simulink library "outp"  (R2021b)
(part 6 of 11)

      link override Signal_Limit/_minval: Value=KOUTP_ACCLevelMem57_enum_minval
      link override Signal_Override/_ovrdflg: Value=KOUTP_ACCLevelMem57_enum_ovrdflg
      link override Signal_Override/_ovrdval: Value=KOUTP_ACCLevelMem57_enum_ovrdval
  VBCM_APMDoorControlSta_flg_Inproc : FVT_lib/outp/OverrideAndLimit  SystemSampleTime=-1  VariantActivationTime=update diagram  Latency=0  AutoFrameSizeCalculation=off
      link override Signal_Limit/_maxval: Value=KOUTP_APMDoorControlSta_flg_maxval
      link override Signal_Limit/_minval: Value=KOUTP_APMDoorControlSta_flg_minval
      link override Signal_Override/_ovrdflg: Value=KOUTP_APMDoorControlSta_flg_ovrdflg
      link override Signal_Override/_ovrdval: Value=KOUTP_APMDoorControlSta_flg_ovrdval
  VBCM_APSOpenPTG_flg_Inproc : FVT_lib/outp/OverrideAndLimit  SystemSampleTime=-1  VariantActivationTime=update diagram  Latency=0  AutoFrameSizeCalculation=off
      link override Signal_Limit/_maxval: Value=KOUTP_APSOpenPTG_flg_maxval
      link override Signal_Limit/_minval: Value=KOUTP_APSOpenPTG_flg_minval
      link override Signal_Override/_ovrdflg: Value=KOUTP_APSOpenPTG_flg_ovrdflg
      link override Signal_Override/_ovrdval: Value=KOUTP_APSOpenPTG_flg_ovrdval
  VBCM_ATCtrl_enum_Inproc : FVT_lib/outp/OverrideAndLimit  SystemSampleTime=-1  VariantActivationTime=update diagram  Latency=0  AutoFrameSizeCalculation=off
      link override Signal_Limit/_maxval: Value=KOUTP_ATCtrl_enum_maxval
      link override Signal_Limit/_minval: Value=KOUTP_ATCtrl_enum_minval
      link override Signal_Override/_ovrdflg: Value=KOUTP_ATCtrl_enum_ovrdflg
      link override Signal_Override/_ovrdval: Value=KOUTP_ATCtrl_enum_ovrdval
  VBCM_AllDoorSW_flg_Inproc : FVT_lib/outp/OverrideAndLimit  SystemSampleTime=-1  VariantActivationTime=update diagram  Latency=0  AutoFrameSizeCalculation=off
      link override Signal_Limit/_maxval: Value=KOUTP_AllDoorSW_flg_maxval
      link override Signal_Limit/_minval: Value=KOUTP_AllDoorSW_flg_minval
      link override Signal_Override/_ovrdflg: Value=KOUTP_AllDoorSW_flg_ovrdflg
      link override Signal_Override/_ovrdval: Value=KOUTP_AllDoorSW_flg_ovrdval
  VBCM_AmbBrightSta_enum_Inproc : FVT_lib/outp/OverrideAndLimit  SystemSampleTime=-1  VariantActivationTime=update diagram  Latency=0  AutoFrameSizeCalculation=off
      link override Signal_Limit/_maxval: Value=KOUTP_AmbBrightSta_enum_maxval
      link override Signal_Limit/_minval: Value=KOUTP_AmbBrightSta_enum_minval
      link override Signal_Override/_ovrdflg: Value=KOUTP_AmbBrightSta_enum_ovrdflg
      link override Signal_Override/_ovrdval: Value=KOUTP_AmbBrightSta_enum_ovrdval
  VBCM_AmbBrightnessSta1_enum_Inproc : FVT_lib/outp/OverrideAndLimit  SystemSampleTime=-1  VariantActivationTime=update diagram  Latency=0  AutoFrameSizeCalculation=off
      link override Signal_Limit/_maxval: Value=KOUTP_AmbBrightnessSta1_enum_maxval
      link override Signal_Limit/_minval: Value=KOUTP_AmbBrightnessSta1_enum_minval
      link override Signal_Override/_ovrdflg: Value=KOUTP_AmbBrightnessSta1_enum_ovrdflg
      link override Signal_Override/_ovrdval: Value=KOUTP_AmbBrightnessSta1_enum_ovrdval
  VBCM_AmbBrightnessSta2_enum_Inproc : FVT_lib/outp/OverrideAndLimit  SystemSampleTime=-1  VariantActivationTime=update diagram  Latency=0  AutoFrameSizeCalculation=off
      link override Signal_Limit/_maxval: Value=KOUTP_AmbBrightnessSta2_enum_maxval
      link override Signal_Limit/_minval: Value=KOUTP_AmbBrightnessSta2_enum_minval
      link override Signal_Override/_ovrdflg: Value=KOUTP_AmbBrightnessSta2_enum_ovrdflg
      link override Signal_Override/_ovrdval: Value=KOUTP_AmbBrightnessSta2_enum_ovrdval
  VBCM_AmbBrightnessSta3_enum_Inproc : FVT_lib/outp/OverrideAndLimit  SystemSampleTime=-1  VariantActivationTime=update diagram  Latency=0  AutoFrameSizeCalculation=off
      link override Signal_Limit/_maxval: Value=KOUTP_AmbBrightnessSta3_enum_maxval
      link override Signal_Limit/_minval: Value=KOUTP_AmbBrightnessSta3_enum_minval
      link override Signal_Override/_ovrdflg: Value=KOUTP_AmbBrightnessSta3_enum_ovrdflg
      link override Signal_Override/_ovrdval: Value=KOUTP_AmbBrightnessSta3_enum_ovrdval
  VBCM_AmbBrightnessSta4_enum_Inproc : FVT_lib/outp/OverrideAndLimit  SystemSampleTime=-1  VariantActivationTime=update diagram  Latency=0  AutoFrameSizeCalculation=off
      link override Signal_Limit/_maxval: Value=KOUTP_AmbBrightnessSta4_enum_maxval
      link override Signal_Limit/_minval: Value=KOUTP_AmbBrightnessSta4_enum_minval
      link override Signal_Override/_ovrdflg: Value=KOUTP_AmbBrightnessSta4_enum_ovrdflg
      link override Signal_Override/_ovrdval: Value=KOUTP_AmbBrightnessSta4_enum_ovrdval
  VBCM_AmbBrightnessSta5_enum_Inproc : FVT_lib/outp/OverrideAndLimit  SystemSampleTime=-1  VariantActivationTime=update diagram  Latency=0  AutoFrameSizeCalculation=off
      link override Signal_Limit/_maxval: Value=KOUTP_AmbBrightnessSta5_enum_maxval
      link override Signal_Limit/_minval: Value=KOUTP_AmbBrightnessSta5_enum_minval
      link override Signal_Override/_ovrdflg: Value=KOUTP_AmbBrightnessSta5_enum_ovrdflg
      link override Signal_Override/_ovrdval: Value=KOUTP_AmbBrightnessSta5_enum_ovrdval
  VBCM_AmbBrightnessSta7_enum_Inproc : FVT_lib/outp/OverrideAndLimit  SystemSampleTime=-1  VariantActivationTime=update diagram  Latency=0  AutoFrameSizeCalculation=off
      link override Signal_Limit/_maxval: Value=KOUTP_AmbBrightnessSta7_enum_maxval
      link override Signal_Limit/_minval: Value=KOUTP_AmbBrightnessSta7_enum_minval
      link override Signal_Override/_ovrdflg: Value=KOUTP_AmbBrightnessSta7_enum_ovrdflg
      link override Signal_Override/_ovrdval: Value=KOUTP_AmbBrightnessSta7_enum_ovrdval
  VBCM_AmbColorSta1_enum_Inproc : FVT_lib/outp/OverrideAndLimit  SystemSampleTime=-1  VariantActivationTime=update diagram  Latency=0  AutoFrameSizeCalculation=off
      link override Signal_Limit/_maxval: Value=KOUTP_AmbColorSta1_enum_maxval
      link override Signal_Limit/_minval: Value=KOUTP_AmbColorSta1_enum_minval
      link override Signal_Override/_ovrdflg: Value=KOUTP_AmbColorSta1_enum_ovrdflg
      link override Signal_Override/_ovrdval: Value=KOUTP_AmbColorSta1_enum_ovrdval
  VBCM_AmbColorSta2_enum_Inproc : FVT_lib/outp/OverrideAndLimit  SystemSampleTime=-1  VariantActivationTime=update diagram  Latency=0  AutoFrameSizeCalculation=off
      link override Signal_Limit/_maxval: Value=KOUTP_AmbColorSta2_enum_maxval
      link override Signal_Limit/_minval: Value=KOUTP_AmbColorSta2_enum_minval
      link override Signal_Override/_ovrdflg: Value=KOUTP_AmbColorSta2_enum_ovrdflg
      link override Signal_Override/_ovrdval: Value=KOUTP_AmbColorSta2_enum_ovrdval
  VBCM_AmbColorSta3_enum_Inproc : FVT_lib/outp/OverrideAndLimit  SystemSampleTime=-1  VariantActivationTime=update diagram  Latency=0  AutoFrameSizeCalculation=off
      link override Signal_Limit/_maxval: Value=KOUTP_AmbColorSta3_enum_maxval
      link override Signal_Limit/_minval: Value=KOUTP_AmbColorSta3_enum_minval
      link override Signal_Override/_ovrdflg: Value=KOUTP_AmbColorSta3_enum_ovrdflg
      link override Signal_Override/_ovrdval: Value=KOUTP_AmbColorSta3_enum_ovrdval
  VBCM_AmbColorSta4_enum_Inproc : FVT_lib/outp/OverrideAndLimit  SystemSampleTime=-1  VariantActivationTime=update diagram  Latency=0  AutoFrameSizeCalculation=off
      link override Signal_Limit/_maxval: Value=KOUTP_AmbColorSta4_enum_maxval
      link override Signal_Limit/_minval: Value=KOUTP_AmbColorSta4_enum_minval
      link override Signal_Override/_ovrdflg: Value=KOUTP_AmbColorSta4_enum_ovrdflg
      link override Signal_Override/_ovrdval: Value=KOUTP_AmbColorSta4_enum_ovrdval
  VBCM_AmbColorSta5_enum_Inproc : FVT_lib/outp/OverrideAndLimit  SystemSampleTime=-1  VariantActivationTime=update diagram  Latency=0  AutoFrameSizeCalculation=off
      link override Signal_Limit/_maxval: Value=KOUTP_AmbColorSta5_enum_maxval
      link override Signal_Limit/_minval: Value=KOUTP_AmbColorSta5_enum_minval
      link override Signal_Override/_ovrdflg: Value=KOUTP_AmbColorSta5_enum_ovrdflg
      link override Signal_Override/_ovrdval: Value=KOUTP_AmbColorSta5_enum_ovrdval
  VBCM_AmbColorSta7_enum_Inproc : FVT_lib/outp/OverrideAndLimit  SystemSampleTime=-1  VariantActivationTime=update diagram  Latency=0  AutoFrameSizeCalculation=off
      link override Signal_Limit/_maxval: Value=KOUTP_AmbColorSta7_enum_maxval
      link override Signal_Limit/_minval: Value=KOUTP_AmbColorSta7_enum_minval
      link override Signal_Override/_ovrdflg: Value=KOUTP_AmbColorSta7_enum_ovrdflg
      link override Signal_Override/_ovrdval: Value=KOUTP_AmbColorSta7_enum_ovrdval
  VBCM_AmbColorSta_enum_Inproc : FVT_lib/outp/OverrideAndLimit  SystemSampleTime=-1  VariantActivationTime=update diagram  Latency=0  AutoFrameSizeCalculation=off
      link override Signal_Limit/_maxval: Value=KOUTP_AmbColorSta_enum_maxval
      link override Signal_Limit/_minval: Value=KOUTP_AmbColorSta_enum_minval
      link override Signal_Override/_ovrdflg: Value=KOUTP_AmbColorSta_enum_ovrdflg
      link override Signal_Override/_ovrdval: Value=KOUTP_AmbColorSta_enum_ovrdval
  VBCM_AmbDimENFlash_enum_Inproc : FVT_lib/outp/OverrideAndLimit  SystemSampleTime=-1  VariantActivationTime=update diagram  Latency=0  AutoFrameSizeCalculation=off
      link override Signal_Limit/_maxval: Value=KOUTP_AmbDimENFlash_enum_maxval
      link override Signal_Limit/_minval: Value=KOUTP_AmbDimENFlash_enum_minval
      link override Signal_Override/_ovrdflg: Value=KOUTP_AmbDimENFlash_enum_ovrdflg
      link override Signal_Override/_ovrdval: Value=KOUTP_AmbDimENFlash_enum_ovrdval
  VBCM_AmbDimEN_flg_Inproc : FVT_lib/outp/OverrideAndLimit  SystemSampleTime=-1  VariantActivationTime=update diagram  Latency=0  AutoFrameSizeCalculation=off
      link override Signal_Limit/_maxval: Value=KOUTP_AmbDimEN_flg_maxval
      link override Signal_Limit/_minval: Value=KOUTP_AmbDimEN_flg_minval
      link override Signal_Override/_ovrdflg: Value=KOUTP_AmbDimEN_flg_ovrdflg
      link override Signal_Override/_ovrdval: Value=KOUTP_AmbDimEN_flg_ovrdval
  VBCM_AmbFunENFlash_enum_Inproc : FVT_lib/outp/OverrideAndLimit  SystemSampleTime=-1  VariantActivationTime=update diagram  Latency=0  AutoFrameSizeCalculation=off
      link override Signal_Limit/_maxval: Value=KOUTP_AmbFunENFlash_enum_maxval
      link override Signal_Limit/_minval: Value=KOUTP_AmbFunENFlash_enum_minval
      link override Signal_Override/_ovrdflg: Value=KOUTP_AmbFunENFlash_enum_ovrdflg
      link override Signal_Override/_ovrdval: Value=KOUTP_AmbFunENFlash_enum_ovrdval
  VBCM_AmbFunEN_flg_Inproc : FVT_lib/outp/OverrideAndLimit  SystemSampleTime=-1  VariantActivationTime=update diagram  Latency=0  AutoFrameSizeCalculation=off
      link override Signal_Limit/_maxval: Value=KOUTP_AmbFunEN_flg_maxval
      link override Signal_Limit/_minval: Value=KOUTP_AmbFunEN_flg_minval
      link override Signal_Override/_ovrdflg: Value=KOUTP_AmbFunEN_flg_ovrdflg
      link override Signal_Override/_ovrdval: Value=KOUTP_AmbFunEN_flg_ovrdval
  VBCM_AmbLightBreath1_enum_Inproc : FVT_lib/outp/OverrideAndLimit  SystemSampleTime=-1  VariantActivationTime=update diagram  Latency=0  AutoFrameSizeCalculation=off
      link override Signal_Limit/_maxval: Value=KOUTP_AmbLightBreath1_enum_maxval
      link override Signal_Limit/_minval: Value=KOUTP_AmbLightBreath1_enum_minval
      link override Signal_Override/_ovrdflg: Value=KOUTP_AmbLightBreath1_enum_ovrdflg
      link override Signal_Override/_ovrdval: Value=KOUTP_AmbLightBreath1_enum_ovrdval
  VBCM_AmbLightBreath2_enum_Inproc : FVT_lib/outp/OverrideAndLimit  SystemSampleTime=-1  VariantActivationTime=update diagram  Latency=0  AutoFrameSizeCalculation=off
      link override Signal_Limit/_maxval: Value=KOUTP_AmbLightBreath2_enum_maxval
      link override Signal_Limit/_minval: Value=KOUTP_AmbLightBreath2_enum_minval
      link override Signal_Override/_ovrdflg: Value=KOUTP_AmbLightBreath2_enum_ovrdflg
      link override Signal_Override/_ovrdval: Value=KOUTP_AmbLightBreath2_enum_ovrdval
  VBCM_AmbLightBreath3_enum_Inproc : FVT_lib/outp/OverrideAndLimit  SystemSampleTime=-1  VariantActivationTime=update diagram  Latency=0  AutoFrameSizeCalculation=off
      link override Signal_Limit/_maxval: Value=KOUTP_AmbLightBreath3_enum_maxval
      link override Signal_Limit/_minval: Value=KOUTP_AmbLightBreath3_enum_minval
      link override Signal_Override/_ovrdflg: Value=KOUTP_AmbLightBreath3_enum_ovrdflg
      link override Signal_Override/_ovrdval: Value=KOUTP_AmbLightBreath3_enum_ovrdval
  VBCM_AmbLightBreath4_enum_Inproc : FVT_lib/outp/OverrideAndLimit  SystemSampleTime=-1  VariantActivationTime=update diagram  Latency=0  AutoFrameSizeCalculation=off
      link override Signal_Limit/_maxval: Value=KOUTP_AmbLightBreath4_enum_maxval
      link override Signal_Limit/_minval: Value=KOUTP_AmbLightBreath4_enum_minval
      link override Signal_Override/_ovrdflg: Value=KOUTP_AmbLightBreath4_enum_ovrdflg
      link override Signal_Override/_ovrdval: Value=KOUTP_AmbLightBreath4_enum_ovrdval
  VBCM_AmbLightBreath5_enum_Inproc : FVT_lib/outp/OverrideAndLimit  SystemSampleTime=-1  VariantActivationTime=update diagram  Latency=0  AutoFrameSizeCalculation=off
      link override Signal_Limit/_maxval: Value=KOUTP_AmbLightBreath5_enum_maxval
      link override Signal_Limit/_minval: Value=KOUTP_AmbLightBreath5_enum_minval
      link override Signal_Override/_ovrdflg: Value=KOUTP_AmbLightBreath5_enum_ovrdflg
      link override Signal_Override/_ovrdval: Value=KOUTP_AmbLightBreath5_enum_ovrdval
  VBCM_AmbLightBreath6_enum_Inproc : FVT_lib/outp/OverrideAndLimit  SystemSampleTime=-1  VariantActivationTime=update diagram  Latency=0  AutoFrameSizeCalculation=off
      link override Signal_Limit/_maxval: Value=KOUTP_AmbLightBreath6_enum_maxval
      link override Signal_Limit/_minval: Value=KOUTP_AmbLightBreath6_enum_minval
      link override Signal_Override/_ovrdflg: Value=KOUTP_AmbLightBreath6_enum_ovrdflg
      link override Signal_Override/_ovrdval: Value=KOUTP_AmbLightBreath6_enum_ovrdval
  VBCM_AmbLightBrightness1_enum_Inproc : FVT_lib/outp/OverrideAndLimit  SystemSampleTime=-1  VariantActivationTime=update diagram  Latency=0  AutoFrameSizeCalculation=off
      link override Signal_Limit/_maxval: Value=KOUTP_AmbLightBrightness1_enum_maxval
      link override Signal_Limit/_minval: Value=KOUTP_AmbLightBrightness1_enum_minval
      link override Signal_Override/_ovrdflg: Value=KOUTP_AmbLightBrightness1_enum_ovrdflg
      link override Signal_Override/_ovrdval: Value=KOUTP_AmbLightBrightness1_enum_ovrdval
  VBCM_AmbLightBrightness2_enum_Inproc : FVT_lib/outp/OverrideAndLimit  SystemSampleTime=-1  VariantActivationTime=update diagram  Latency=0  AutoFrameSizeCalculation=off
      link override Signal_Limit/_maxval: Value=KOUTP_AmbLightBrightness2_enum_maxval
      link override Signal_Limit/_minval: Value=KOUTP_AmbLightBrightness2_enum_minval
      link override Signal_Override/_ovrdflg: Value=KOUTP_AmbLightBrightness2_enum_ovrdflg
      link override Signal_Override/_ovrdval: Value=KOUTP_AmbLightBrightness2_enum_ovrdval
  VBCM_AmbLightBrightness3_enum_Inproc : FVT_lib/outp/OverrideAndLimit  SystemSampleTime=-1  VariantActivationTime=update diagram  Latency=0  AutoFrameSizeCalculation=off
      link override Signal_Limit/_maxval: Value=KOUTP_AmbLightBrightness3_enum_maxval
      link override Signal_Limit/_minval: Value=KOUTP_AmbLightBrightness3_enum_minval
      link override Signal_Override/_ovrdflg: Value=KOUTP_AmbLightBrightness3_enum_ovrdflg
      link override Signal_Override/_ovrdval: Value=KOUTP_AmbLightBrightness3_enum_ovrdval
  VBCM_AmbLightBrightness4_enum_Inproc : FVT_lib/outp/OverrideAndLimit  SystemSampleTime=-1  VariantActivationTime=update diagram  Latency=0  AutoFrameSizeCalculation=off
      link override Signal_Limit/_maxval: Value=KOUTP_AmbLightBrightness4_enum_maxval
      link override Signal_Limit/_minval: Value=KOUTP_AmbLightBrightness4_enum_minval
      link override Signal_Override/_ovrdflg: Value=KOUTP_AmbLightBrightness4_enum_ovrdflg
      link override Signal_Override/_ovrdval: Value=KOUTP_AmbLightBrightness4_enum_ovrdval
  VBCM_AmbLightBrightness5_enum_Inproc : FVT_lib/outp/OverrideAndLimit  SystemSampleTime=-1  VariantActivationTime=update diagram  Latency=0  AutoFrameSizeCalculation=off
      link override Signal_Limit/_maxval: Value=KOUTP_AmbLightBrightness5_enum_maxval
      link override Signal_Limit/_minval: Value=KOUTP_AmbLightBrightness5_enum_minval
      link override Signal_Override/_ovrdflg: Value=KOUTP_AmbLightBrightness5_enum_ovrdflg
      link override Signal_Override/_ovrdval: Value=KOUTP_AmbLightBrightness5_enum_ovrdval
  VBCM_AmbLightBrightness6_enum_Inproc : FVT_lib/outp/OverrideAndLimit  SystemSampleTime=-1  VariantActivationTime=update diagram  Latency=0  AutoFrameSizeCalculation=off
      link override Signal_Limit/_maxval: Value=KOUTP_AmbLightBrightness6_enum_maxval
      link override Signal_Limit/_minval: Value=KOUTP_AmbLightBrightness6_enum_minval
      link override Signal_Override/_ovrdflg: Value=KOUTP_AmbLightBrightness6_enum_ovrdflg
      link override Signal_Override/_ovrdval: Value=KOUTP_AmbLightBrightness6_enum_ovrdval
  VBCM_AmbLightColor1_enum_Inproc : FVT_lib/outp/OverrideAndLimit  SystemSampleTime=-1  VariantActivationTime=update diagram  Latency=0  AutoFrameSizeCalculation=off
      link override Signal_Limit/_maxval: Value=KOUTP_AmbLightColor1_enum_maxval
      link override Signal_Limit/_minval: Value=KOUTP_AmbLightColor1_enum_minval
      link override Signal_Override/_ovrdflg: Value=KOUTP_AmbLightColor1_enum_ovrdflg
      link override Signal_Override/_ovrdval: Value=KOUTP_AmbLightColor1_enum_ovrdval
  VBCM_AmbLightColor2_enum_Inproc : FVT_lib/outp/OverrideAndLimit  SystemSampleTime=-1  VariantActivationTime=update diagram  Latency=0  AutoFrameSizeCalculation=off
      link override Signal_Limit/_maxval: Value=KOUTP_AmbLightColor2_enum_maxval
      link override Signal_Limit/_minval: Value=KOUTP_AmbLightColor2_enum_minval
      link override Signal_Override/_ovrdflg: Value=KOUTP_AmbLightColor2_enum_ovrdflg
      link override Signal_Override/_ovrdval: Value=KOUTP_AmbLightColor2_enum_ovrdval
  VBCM_AmbLightColor3_enum_Inproc : FVT_lib/outp/OverrideAndLimit  SystemSampleTime=-1  VariantActivationTime=update diagram  Latency=0  AutoFrameSizeCalculation=off
      link override Signal_Limit/_maxval: Value=KOUTP_AmbLightColor3_enum_maxval
      link override Signal_Limit/_minval: Value=KOUTP_AmbLightColor3_enum_minval
      link override Signal_Override/_ovrdflg: Value=KOUTP_AmbLightColor3_enum_ovrdflg
      link override Signal_Override/_ovrdval: Value=KOUTP_AmbLightColor3_enum_ovrdval
  VBCM_AmbLightColor4_enum_Inproc : FVT_lib/outp/OverrideAndLimit  SystemSampleTime=-1  VariantActivationTime=update diagram  Latency=0  AutoFrameSizeCalculation=off
      link override Signal_Limit/_maxval: Value=KOUTP_AmbLightColor4_enum_maxval
      link override Signal_Limit/_minval: Value=KOUTP_AmbLightColor4_enum_minval
      link override Signal_Override/_ovrdflg: Value=KOUTP_AmbLightColor4_enum_ovrdflg
      link override Signal_Override/_ovrdval: Value=KOUTP_AmbLightColor4_enum_ovrdval
  VBCM_AmbLightColor5_enum_Inproc : FVT_lib/outp/OverrideAndLimit  SystemSampleTime=-1  VariantActivationTime=update diagram  Latency=0  AutoFrameSizeCalculation=off
      link override Signal_Limit/_maxval: Value=KOUTP_AmbLightColor5_enum_maxval
      link override Signal_Limit/_minval: Value=KOUTP_AmbLightColor5_enum_minval
      link override Signal_Override/_ovrdflg: Value=KOUTP_AmbLightColor5_enum_ovrdflg
      link override Signal_Override/_ovrdval: Value=KOUTP_AmbLightColor5_enum_ovrdval
  VBCM_AmbLightColor6_enum_Inproc : FVT_lib/outp/OverrideAndLimit  SystemSampleTime=-1  VariantActivationTime=update diagram  Latency=0  AutoFrameSizeCalculation=off
      link override Signal_Limit/_maxval: Value=KOUTP_AmbLightColor6_enum_maxval
      link override Signal_Limit/_minval: Value=KOUTP_AmbLightColor6_enum_minval
      link override Signal_Override/_ovrdflg: Value=KOUTP_AmbLightColor6_enum_ovrdflg
      link override Signal_Override/_ovrdval: Value=KOUTP_AmbLightColor6_enum_ovrdval
  VBCM_AmbLinkDriStaFlash_enum_Inproc : FVT_lib/outp/OverrideAndLimit  SystemSampleTime=-1  VariantActivationTime=update diagram  Latency=0  AutoFrameSizeCalculation=off
      link override Signal_Limit/_maxval: Value=KOUTP_AmbLinkDriStaFlash_enum_maxval
      link override Signal_Limit/_minval: Value=KOUTP_AmbLinkDriStaFlash_enum_minval
      link override Signal_Override/_ovrdflg: Value=KOUTP_AmbLinkDriStaFlash_enum_ovrdflg
      link override Signal_Override/_ovrdval: Value=KOUTP_AmbLinkDriStaFlash_enum_ovrdval
  VBCM_AmbLinkDriSta_flg_Inproc : FVT_lib/outp/OverrideAndLimit  SystemSampleTime=-1  VariantActivationTime=update diagram  Latency=0  AutoFrameSizeCalculation=off
      link override Signal_Limit/_maxval: Value=KOUTP_AmbLinkDriSta_flg_maxval
      link override Signal_Limit/_minval: Value=KOUTP_AmbLinkDriSta_flg_minval
      link override Signal_Override/_ovrdflg: Value=KOUTP_AmbLinkDriSta_flg_ovrdflg
      link override Signal_Override/_ovrdval: Value=KOUTP_AmbLinkDriSta_flg_ovrdval
  VBCM_AmbODAENFlash_enum_Inproc : FVT_lib/outp/OverrideAndLimit  SystemSampleTime=-1  VariantActivationTime=update diagram  Latency=0  AutoFrameSizeCalculation=off
      link override Signal_Limit/_maxval: Value=KOUTP_AmbODAENFlash_enum_maxval
      link override Signal_Limit/_minval: Value=KOUTP_AmbODAENFlash_enum_minval
      link override Signal_Override/_ovrdflg: Value=KOUTP_AmbODAENFlash_enum_ovrdflg
      link override Signal_Override/_ovrdval: Value=KOUTP_AmbODAENFlash_enum_ovrdval
  VBCM_AmbODAEN_flg_Inproc : FVT_lib/outp/OverrideAndLimit  SystemSampleTime=-1  VariantActivationTime=update diagram  Latency=0  AutoFrameSizeCalculation=off
      link override Signal_Limit/_maxval: Value=KOUTP_AmbODAEN_flg_maxval
      link override Signal_Limit/_minval: Value=KOUTP_AmbODAEN_flg_minval
      link override Signal_Override/_ovrdflg: Value=KOUTP_AmbODAEN_flg_ovrdflg
      link override Signal_Override/_ovrdval: Value=KOUTP_AmbODAEN_flg_ovrdval
  VBCM_AmbPwrWarnENFlash_enum_Inproc : FVT_lib/outp/OverrideAndLimit  SystemSampleTime=-1  VariantActivationTime=update diagram  Latency=0  AutoFrameSizeCalculation=off
      link override Signal_Limit/_maxval: Value=KOUTP_AmbPwrWarnENFlash_enum_maxval
      link override Signal_Limit/_minval: Value=KOUTP_AmbPwrWarnENFlash_enum_minval
      link override Signal_Override/_ovrdflg: Value=KOUTP_AmbPwrWarnENFlash_enum_ovrdflg
      link override Signal_Override/_ovrdval: Value=KOUTP_AmbPwrWarnENFlash_enum_ovrdval
  VBCM_AmbPwrWarnEN_flg_Inproc : FVT_lib/outp/OverrideAndLimit  SystemSampleTime=-1  VariantActivationTime=update diagram  Latency=0  AutoFrameSizeCalculation=off
      link override Signal_Limit/_maxval: Value=KOUTP_AmbPwrWarnEN_flg_maxval
      link override Signal_Limit/_minval: Value=KOUTP_AmbPwrWarnEN_flg_minval
      link override Signal_Override/_ovrdflg: Value=KOUTP_AmbPwrWarnEN_flg_ovrdflg
      link override Signal_Override/_ovrdval: Value=KOUTP_AmbPwrWarnEN_flg_ovrdval
  VBCM_AmbWelENFlash_enum_Inproc : FVT_lib/outp/OverrideAndLimit  SystemSampleTime=-1  VariantActivationTime=update diagram  Latency=0  AutoFrameSizeCalculation=off
      link override Signal_Limit/_maxval: Value=KOUTP_AmbWelENFlash_enum_maxval
      link override Signal_Limit/_minval: Value=KOUTP_AmbWelENFlash_enum_minval
      link override Signal_Override/_ovrdflg: Value=KOUTP_AmbWelENFlash_enum_ovrdflg
      link override Signal_Override/_ovrdval: Value=KOUTP_AmbWelENFlash_enum_ovrdval
  VBCM_AmbWelEN_flg_Inproc : FVT_lib/outp/OverrideAndLimit  SystemSampleTime=-1  VariantActivationTime=update diagram  Latency=0  AutoFrameSizeCalculation=off
      link override Signal_Limit/_maxval: Value=KOUTP_AmbWelEN_flg_maxval
      link override Signal_Limit/_minval: Value=KOUTP_AmbWelEN_flg_minval
      link override Signal_Override/_ovrdflg: Value=KOUTP_AmbWelEN_flg_ovrdflg
      link override Signal_Override/_ovrdval: Value=KOUTP_AmbWelEN_flg_ovrdval
  VBCM_AntitheftSeatFlod_flg_Inproc : FVT_lib/outp/OverrideAndLimit  SystemSampleTime=-1  VariantActivationTime=update diagram  Latency=0  AutoFrameSizeCalculation=off
      link override Signal_Limit/_maxval: Value=KOUTP_AntitheftSeatFlod_flg_maxval
      link override Signal_Limit/_minval: Value=KOUTP_AntitheftSeatFlod_flg_minval
      link override Signal_Override/_ovrdflg: Value=KOUTP_AntitheftSeatFlod_flg_ovrdflg
      link override Signal_Override/_ovrdval: Value=KOUTP_AntitheftSeatFlod_flg_ovrdval
  VBCM_AntitheftSta_enum_Inproc : FVT_lib/outp/OverrideAndLimit  SystemSampleTime=-1  VariantActivationTime=update diagram  Latency=0  AutoFrameSizeCalculation=off
      link override Signal_Limit/_maxval: Value=KOUTP_AntitheftSta_enum_maxval
      link override Signal_Limit/_minval: Value=KOUTP_AntitheftSta_enum_minval
      link override Signal_Override/_ovrdflg: Value=KOUTP_AntitheftSta_enum_ovrdflg
      link override Signal_Override/_ovrdval: Value=KOUTP_AntitheftSta_enum_ovrdval
  VBCM_AutoLockMem_enum_Inproc : FVT_lib/outp/OverrideAndLimit  SystemSampleTime=-1  VariantActivationTime=update diagram  Latency=0  AutoFrameSizeCalculation=off
      link override Signal_Limit/_maxval: Value=KOUTP_AutoLockMem_enum_maxval
      link override Signal_Limit/_minval: Value=KOUTP_AutoLockMem_enum_minval
      link override Signal_Override/_ovrdflg: Value=KOUTP_AutoLockMem_enum_ovrdflg
      link override Signal_Override/_ovrdval: Value=KOUTP_AutoLockMem_enum_ovrdval
  VBCM_AutoLockSta_flg_Inproc : FVT_lib/outp/OverrideAndLimit  SystemSampleTime=-1  VariantActivationTime=update diagram  Latency=0  AutoFrameSizeCalculation=off
      link override Signal_Limit/_maxval: Value=KOUTP_AutoLockSta_flg_maxval
      link override Signal_Limit/_minval: Value=KOUTP_AutoLockSta_flg_minval
      link override Signal_Override/_ovrdflg: Value=KOUTP_AutoLockSta_flg_ovrdflg
      link override Signal_Override/_ovrdval: Value=KOUTP_AutoLockSta_flg_ovrdval
  VBCM_AutoUnlockMem_enum_Inproc : FVT_lib/outp/OverrideAndLimit  SystemSampleTime=-1  VariantActivationTime=update diagram  Latency=0  AutoFrameSizeCalculation=off
      link override Signal_Limit/_maxval: Value=KOUTP_AutoUnlockMem_enum_maxval
      link override Signal_Limit/_minval: Value=KOUTP_AutoUnlockMem_enum_minval
      link override Signal_Override/_ovrdflg: Value=KOUTP_AutoUnlockMem_enum_ovrdflg
      link override Signal_Override/_ovrdval: Value=KOUTP_AutoUnlockMem_enum_ovrdval
  VBCM_AutoUnlockSta_flg_Inproc : FVT_lib/outp/OverrideAndLimit  SystemSampleTime=-1  VariantActivationTime=update diagram  Latency=0  AutoFrameSizeCalculation=off
      link override Signal_Limit/_maxval: Value=KOUTP_AutoUnlockSta_flg_maxval
      link override Signal_Limit/_minval: Value=KOUTP_AutoUnlockSta_flg_minval
      link override Signal_Override/_ovrdflg: Value=KOUTP_AutoUnlockSta_flg_ovrdflg
      link override Signal_Override/_ovrdval: Value=KOUTP_AutoUnlockSta_flg_ovrdval
  VBCM_AutoWipHSpdENSta_flg_Inproc : FVT_lib/outp/OverrideAndLimit  SystemSampleTime=-1  VariantActivationTime=update diagram  Latency=0  AutoFrameSizeCalculation=off
      link override Signal_Limit/_maxval: Value=KOUTP_AutoWipHSpdENSta_flg_maxval
      link override Signal_Limit/_minval: Value=KOUTP_AutoWipHSpdENSta_flg_minval
      link override Signal_Override/_ovrdflg: Value=KOUTP_AutoWipHSpdENSta_flg_ovrdflg
      link override Signal_Override/_ovrdval: Value=KOUTP_AutoWipHSpdENSta_flg_ovrdval
  VBCM_BCMBuzzerReq_flg_Inproc : FVT_lib/outp/OverrideAndLimit  SystemSampleTime=-1  VariantActivationTime=update diagram  Latency=0  AutoFrameSizeCalculation=off
      link override Signal_Limit/_maxval: Value=KOUTP_BCMBuzzerReq_flg_maxval
      link override Signal_Limit/_minval: Value=KOUTP_BCMBuzzerReq_flg_minval
      link override Signal_Override/_ovrdflg: Value=KOUTP_BCMBuzzerReq_flg_ovrdflg
      link override Signal_Override/_ovrdval: Value=KOUTP_BCMBuzzerReq_flg_ovrdval
  VBCM_BCMDoorLockSta_flg_Inproc : FVT_lib/outp/OverrideAndLimit  SystemSampleTime=-1  VariantActivationTime=update diagram  Latency=0  AutoFrameSizeCalculation=off
      link override Signal_Limit/_maxval: Value=KOUTP_BCMDoorLockSta_flg_maxval
      link override Signal_Limit/_minval: Value=KOUTP_BCMDoorLockSta_flg_minval
      link override Signal_Override/_ovrdflg: Value=KOUTP_BCMDoorLockSta_flg_ovrdflg
      link override Signal_Override/_ovrdval: Value=KOUTP_BCMDoorLockSta_flg_ovrdval
  VBCM_BrakeLamp_flg_Inproc : FVT_lib/outp/OverrideAndLimit  SystemSampleTime=-1  VariantActivationTime=update diagram  Latency=0  AutoFrameSizeCalculation=off
      link override Signal_Limit/_maxval: Value=KOUTP_BrakeLamp_flg_maxval
      link override Signal_Limit/_minval: Value=KOUTP_BrakeLamp_flg_minval
      link override Signal_Override/_ovrdflg: Value=KOUTP_BrakeLamp_flg_ovrdflg
      link override Signal_Override/_ovrdval: Value=KOUTP_BrakeLamp_flg_ovrdval
  VBCM_CLWinLockDrStaMem_enum_Inproc : FVT_lib/outp/OverrideAndLimit  SystemSampleTime=-1  VariantActivationTime=update diagram  Latency=0  AutoFrameSizeCalculation=off
      link override Signal_Limit/_maxval: Value=KOUTP_CLWinLockDrStaMem_enum_maxval
      link override Signal_Limit/_minval: Value=KOUTP_CLWinLockDrStaMem_enum_minval
      link override Signal_Override/_ovrdflg: Value=KOUTP_CLWinLockDrStaMem_enum_ovrdflg
      link override Signal_Override/_ovrdval: Value=KOUTP_CLWinLockDrStaMem_enum_ovrdval
  VBCM_CLWinLockDrSta_flg_Inproc : FVT_lib/outp/OverrideAndLimit  SystemSampleTime=-1  VariantActivationTime=update diagram  Latency=0  AutoFrameSizeCalculation=off
      link override Signal_Limit/_maxval: Value=KOUTP_CLWinLockDrSta_flg_maxval
      link override Signal_Limit/_minval: Value=KOUTP_CLWinLockDrSta_flg_minval
      link override Signal_Override/_ovrdflg: Value=KOUTP_CLWinLockDrSta_flg_ovrdflg
      link override Signal_Override/_ovrdval: Value=KOUTP_CLWinLockDrSta_flg_ovrdval
  VBCM_CTDCtrl_enum_Inproc : FVT_lib/outp/OverrideAndLimit  SystemSampleTime=-1  VariantActivationTime=update diagram  Latency=0  AutoFrameSizeCalculation=off
      link override Signal_Limit/_maxval: Value=KOUTP_CTDCtrl_enum_maxval
      link override Signal_Limit/_minval: Value=KOUTP_CTDCtrl_enum_minval
      link override Signal_Override/_ovrdflg: Value=KOUTP_CTDCtrl_enum_ovrdflg
      link override Signal_Override/_ovrdval: Value=KOUTP_CTDCtrl_enum_ovrdval
  VBCM_CTDLockSW_flg_Inproc : FVT_lib/outp/OverrideAndLimit  SystemSampleTime=-1  VariantActivationTime=update diagram  Latency=0  AutoFrameSizeCalculation=off
      link override Signal_Limit/_maxval: Value=KOUTP_CTDLockSW_flg_maxval
      link override Signal_Limit/_minval: Value=KOUTP_CTDLockSW_flg_minval
      link override Signal_Override/_ovrdflg: Value=KOUTP_CTDLockSW_flg_ovrdflg
      link override Signal_Override/_ovrdval: Value=KOUTP_CTDLockSW_flg_ovrdval
  VBCM_CountAlarm_enum_Inproc : FVT_lib/outp/OverrideAndLimit  SystemSampleTime=-1  VariantActivationTime=update diagram  Latency=0  AutoFrameSizeCalculation=off
      link override Signal_Limit/_maxval: Value=KOUTP_CountAlarm_enum_maxval
      link override Signal_Limit/_minval: Value=KOUTP_CountAlarm_enum_minval
      link override Signal_Override/_ovrdflg: Value=KOUTP_CountAlarm_enum_ovrdflg
      link override Signal_Override/_ovrdval: Value=KOUTP_CountAlarm_enum_ovrdval
  VBCM_CrashDetd_flg_Inproc : FVT_lib/outp/OverrideAndLimit  SystemSampleTime=-1  VariantActivationTime=update diagram  Latency=0  AutoFrameSizeCalculation=off
      link override Signal_Limit/_maxval: Value=KOUTP_CrashDetd_flg_maxval
      link override Signal_Limit/_minval: Value=KOUTP_CrashDetd_flg_minval
      link override Signal_Override/_ovrdflg: Value=KOUTP_CrashDetd_flg_ovrdflg
      link override Signal_Override/_ovrdval: Value=KOUTP_CrashDetd_flg_ovrdval
  VBCM_DimSwSta_flg_Inproc : FVT_lib/outp/OverrideAndLimit  SystemSampleTime=-1  VariantActivationTime=update diagram  Latency=0  AutoFrameSizeCalculation=off
      link override Signal_Limit/_maxval: Value=KOUTP_DimSwSta_flg_maxval
      link override Signal_Limit/_minval: Value=KOUTP_DimSwSta_flg_minval
      link override Signal_Override/_ovrdflg: Value=KOUTP_DimSwSta_flg_ovrdflg
      link override Signal_Override/_ovrdval: Value=KOUTP_DimSwSta_flg_ovrdval
  VBCM_DimmerEN_flg_Inproc : FVT_lib/outp/OverrideAndLimit  SystemSampleTime=-1  VariantActivationTime=update diagram  Latency=0  AutoFrameSizeCalculation=off
      link override Signal_Limit/_maxval: Value=KOUTP_DimmerEN_flg_maxval
      link override Signal_Limit/_minval: Value=KOUTP_DimmerEN_flg_minval
      link override Signal_Override/_ovrdflg: Value=KOUTP_DimmerEN_flg_ovrdflg
      link override Signal_Override/_ovrdval: Value=KOUTP_DimmerEN_flg_ovrdval
  VBCM_Dimmer_pct_Inproc : FVT_lib/outp/OverrideAndLimit  SystemSampleTime=-1  VariantActivationTime=update diagram  Latency=0  AutoFrameSizeCalculation=off
      link override Signal_Limit/_maxval: Value=KOUTP_Dimmer_pct_maxval
      link override Signal_Limit/_minval: Value=KOUTP_Dimmer_pct_minval
      link override Signal_Override/_ovrdflg: Value=KOUTP_Dimmer_pct_ovrdflg
      link override Signal_Override/_ovrdval: Value=KOUTP_Dimmer_pct_ovrdval
  VBCM_DoorLockIND_flg_Inproc : FVT_lib/outp/OverrideAndLimit  SystemSampleTime=-1  VariantActivationTime=update diagram  Latency=0  AutoFrameSizeCalculation=off
      link override Signal_Limit/_maxval: Value=KOUTP_DoorLockIND_flg_maxval
      link override Signal_Limit/_minval: Value=KOUTP_DoorLockIND_flg_minval
      link override Signal_Override/_ovrdflg: Value=KOUTP_DoorLockIND_flg_ovrdflg
      link override Signal_Override/_ovrdval: Value=KOUTP_DoorLockIND_flg_ovrdval
  VBCM_DrDoorSW_flg_Inproc : FVT_lib/outp/OverrideAndLimit  SystemSampleTime=-1  VariantActivationTime=update diagram  Latency=0  AutoFrameSizeCalculation=off
      link override Signal_Limit/_maxval: Value=KOUTP_DrDoorSW_flg_maxval
      link override Signal_Limit/_minval: Value=KOUTP_DrDoorSW_flg_minval
      link override Signal_Override/_ovrdflg: Value=KOUTP_DrDoorSW_flg_ovrdflg
      link override Signal_Override/_ovrdval: Value=KOUTP_DrDoorSW_flg_ovrdval
  VBCM_DrRWdwCtrlCmd_pct_Inproc : FVT_lib/outp/OverrideAndLimit  SystemSampleTime=-1  VariantActivationTime=update diagram  Latency=0  AutoFrameSizeCalculation=off
      link override Signal_Limit/_maxval: Value=KOUTP_DrRWdwCtrlCmd_pct_maxval
      link override Signal_Limit/_minval: Value=KOUTP_DrRWdwCtrlCmd_pct_minval
      link override Signal_Override/_ovrdflg: Value=KOUTP_DrRWdwCtrlCmd_pct_ovrdflg
      link override Signal_Override/_ovrdval: Value=KOUTP_DrRWdwCtrlCmd_pct_ovrdval
  VBCM_DrRWdwReqAP_enum_Inproc : FVT_lib/outp/OverrideAndLimit  SystemSampleTime=-1  VariantActivationTime=update diagram  Latency=0  AutoFrameSizeCalculation=off
      link override Signal_Limit/_maxval: Value=KOUTP_DrRWdwReqAP_enum_maxval
      link override Signal_Limit/_minval: Value=KOUTP_DrRWdwReqAP_enum_minval
      link override Signal_Override/_ovrdflg: Value=KOUTP_DrRWdwReqAP_enum_ovrdflg
      link override Signal_Override/_ovrdval: Value=KOUTP_DrRWdwReqAP_enum_ovrdval
  VBCM_DrvWdwCtrlCmd_pct_Inproc : FVT_lib/outp/OverrideAndLimit  SystemSampleTime=-1  VariantActivationTime=update diagram  Latency=0  AutoFrameSizeCalculation=off
      link override Signal_Limit/_maxval: Value=KOUTP_DrvWdwCtrlCmd_pct_maxval
      link override Signal_Limit/_minval: Value=KOUTP_DrvWdwCtrlCmd_pct_minval
      link override Signal_Override/_ovrdflg: Value=KOUTP_DrvWdwCtrlCmd_pct_ovrdflg
      link override Signal_Override/_ovrdval: Value=KOUTP_DrvWdwCtrlCmd_pct_ovrdval
  VBCM_DrvWdwReqAP_enum_Inproc : FVT_lib/outp/OverrideAndLimit  SystemSampleTime=-1  VariantActivationTime=update diagram  Latency=0  AutoFrameSizeCalculation=off
      link override Signal_Limit/_maxval: Value=KOUTP_DrvWdwReqAP_enum_maxval
      link override Signal_Limit/_minval: Value=KOUTP_DrvWdwReqAP_enum_minval
      link override Signal_Override/_ovrdflg: Value=KOUTP_DrvWdwReqAP_enum_ovrdflg
      link override Signal_Override/_ovrdval: Value=KOUTP_DrvWdwReqAP_enum_ovrdval
  VBCM_FDHandleCmd_enum_Inproc : FVT_lib/outp/OverrideAndLimit  SystemSampleTime=-1  VariantActivationTime=update diagram  Latency=0  AutoFrameSizeCalculation=off
      link override Signal_Limit/_maxval: Value=KOUTP_FDHandleCmd_enum_maxval
      link override Signal_Limit/_minval: Value=KOUTP_FDHandleCmd_enum_minval
      link override Signal_Override/_ovrdflg: Value=KOUTP_FDHandleCmd_enum_ovrdflg
      link override Signal_Override/_ovrdval: Value=KOUTP_FDHandleCmd_enum_ovrdval
  VBCM_FDLHandleLampCmd_flg_Inproc : FVT_lib/outp/OverrideAndLimit  SystemSampleTime=-1  VariantActivationTime=update diagram  Latency=0  AutoFrameSizeCalculation=off
      link override Signal_Limit/_maxval: Value=KOUTP_FDLHandleLampCmd_flg_maxval
      link override Signal_Limit/_minval: Value=KOUTP_FDLHandleLampCmd_flg_minval
      link override Signal_Override/_ovrdflg: Value=KOUTP_FDLHandleLampCmd_flg_ovrdflg
      link override Signal_Override/_ovrdval: Value=KOUTP_FDLHandleLampCmd_flg_ovrdval
  VBCM_FDRHandleLampCmd_flg_Inproc : FVT_lib/outp/OverrideAndLimit  SystemSampleTime=-1  VariantActivationTime=update diagram  Latency=0  AutoFrameSizeCalculation=off
      link override Signal_Limit/_maxval: Value=KOUTP_FDRHandleLampCmd_flg_maxval
      link override Signal_Limit/_minval: Value=KOUTP_FDRHandleLampCmd_flg_minval
      link override Signal_Override/_ovrdflg: Value=KOUTP_FDRHandleLampCmd_flg_ovrdflg
      link override Signal_Override/_ovrdval: Value=KOUTP_FDRHandleLampCmd_flg_ovrdval
  VBCM_FWasSwSta_enum_Inproc : FVT_lib/outp/OverrideAndLimit  SystemSampleTime=-1  VariantActivationTime=update diagram  Latency=0  AutoFrameSizeCalculation=off
      link override Signal_Limit/_maxval: Value=KOUTP_FWasSwSta_enum_maxval
      link override Signal_Limit/_minval: Value=KOUTP_FWasSwSta_enum_minval
      link override Signal_Override/_ovrdflg: Value=KOUTP_FWasSwSta_enum_ovrdflg
      link override Signal_Override/_ovrdval: Value=KOUTP_FWasSwSta_enum_ovrdval
  VBCM_FWipSwSta_enum_Inproc : FVT_lib/outp/OverrideAndLimit  SystemSampleTime=-1  VariantActivationTime=update diagram  Latency=0  AutoFrameSizeCalculation=off
      link override Signal_Limit/_maxval: Value=KOUTP_FWipSwSta_enum_maxval
      link override Signal_Limit/_minval: Value=KOUTP_FWipSwSta_enum_minval
      link override Signal_Override/_ovrdflg: Value=KOUTP_FWipSwSta_enum_ovrdflg
      link override Signal_Override/_ovrdval: Value=KOUTP_FWipSwSta_enum_ovrdval
  VBCM_FollowMeENFunSta_flg_Inproc : FVT_lib/outp/OverrideAndLimit  SystemSampleTime=-1  VariantActivationTime=update diagram  Latency=0  AutoFrameSizeCalculation=off
      link override Signal_Limit/_maxval: Value=KOUTP_FollowMeENFunSta_flg_maxval
      link override Signal_Limit/_minval: Value=KOUTP_FollowMeENFunSta_flg_minval
      link override Signal_Override/_ovrdflg: Value=KOUTP_FollowMeENFunSta_flg_ovrdflg
      link override Signal_Override/_ovrdval: Value=KOUTP_FollowMeENFunSta_flg_ovrdval
  VBCM_FollowMeENMem_enum_Inproc : FVT_lib/outp/OverrideAndLimit  SystemSampleTime=-1  VariantActivationTime=update diagram  Latency=0  AutoFrameSizeCalculation=off
      link override Signal_Limit/_maxval: Value=KOUTP_FollowMeENMem_enum_maxval
      link override Signal_Limit/_minval: Value=KOUTP_FollowMeENMem_enum_minval
      link override Signal_Override/_ovrdflg: Value=KOUTP_FollowMeENMem_enum_ovrdflg
      link override Signal_Override/_ovrdval: Value=KOUTP_FollowMeENMem_enum_ovrdval
  VBCM_FollowMe_flg_Inproc : FVT_lib/outp/OverrideAndLimit  SystemSampleTime=-1  VariantActivationTime=update diagram  Latency=0  AutoFrameSizeCalculation=off
      link override Signal_Limit/_maxval: Value=KOUTP_FollowMe_flg_maxval
      link override Signal_Limit/_minval: Value=KOUTP_FollowMe_flg_minval
      link override Signal_Override/_ovrdflg: Value=KOUTP_FollowMe_flg_ovrdflg
      link override Signal_Override/_ovrdval: Value=KOUTP_FollowMe_flg_ovrdval
  VBCM_FrChargingDoorCtrl_enum_Inproc : FVT_lib/outp/OverrideAndLimit  SystemSampleTime=-1  VariantActivationTime=update diagram  Latency=0  AutoFrameSizeCalculation=off
      link override Signal_Limit/_maxval: Value=KOUTP_FrChargingDoorCtrl_enum_maxval
      link override Signal_Limit/_minval: Value=KOUTP_FrChargingDoorCtrl_enum_minval
      link override Signal_Override/_ovrdflg: Value=KOUTP_FrChargingDoorCtrl_enum_ovrdflg
      link override Signal_Override/_ovrdval: Value=KOUTP_FrChargingDoorCtrl_enum_ovrdval
  VBCM_FrWiperH_flg_Inproc : FVT_lib/outp/OverrideAndLimit  SystemSampleTime=-1  VariantActivationTime=update diagram  Latency=0  AutoFrameSizeCalculation=off
      link override Signal_Limit/_maxval: Value=KOUTP_FrWiperH_flg_maxval
      link override Signal_Limit/_minval: Value=KOUTP_FrWiperH_flg_minval
      link override Signal_Override/_ovrdflg: Value=KOUTP_FrWiperH_flg_ovrdflg
      link override Signal_Override/_ovrdval: Value=KOUTP_FrWiperH_flg_ovrdval
  VBCM_FrWiperL_flg_Inproc : FVT_lib/outp/OverrideAndLimit  SystemSampleTime=-1  VariantActivationTime=update diagram  Latency=0  AutoFrameSizeCalculation=off
      link override Signal_Limit/_maxval: Value=KOUTP_FrWiperL_flg_maxval
      link override Signal_Limit/_minval: Value=KOUTP_FrWiperL_flg_minval
      link override Signal_Override/_ovrdflg: Value=KOUTP_FrWiperL_flg_ovrdflg
      link override Signal_Override/_ovrdval: Value=KOUTP_FrWiperL_flg_ovrdval
  VBCM_FuelDoorPos_flg_Inproc : FVT_lib/outp/OverrideAndLimit  SystemSampleTime=-1  VariantActivationTime=update diagram  Latency=0  AutoFrameSizeCalculation=off
      link override Signal_Limit/_maxval: Value=KOUTP_FuelDoorPos_flg_maxval
      link override Signal_Limit/_minval: Value=KOUTP_FuelDoorPos_flg_minval
      link override Signal_Override/_ovrdflg: Value=KOUTP_FuelDoorPos_flg_ovrdflg
      link override Signal_Override/_ovrdval: Value=KOUTP_FuelDoorPos_flg_ovrdval
  VBCM_HBeamADB_flg_Inproc : FVT_lib/outp/OverrideAndLimit  SystemSampleTime=-1  VariantActivationTime=update diagram  Latency=0  AutoFrameSizeCalculation=off
      link override Signal_Limit/_maxval: Value=KOUTP_HBeamADB_flg_maxval
      link override Signal_Limit/_minval: Value=KOUTP_HBeamADB_flg_minval
      link override Signal_Override/_ovrdflg: Value=KOUTP_HBeamADB_flg_ovrdflg
      link override Signal_Override/_ovrdval: Value=KOUTP_HBeamADB_flg_ovrdval
  VBCM_HBeam_flg_Inproc : FVT_lib/outp/OverrideAndLimit  SystemSampleTime=-1  VariantActivationTime=update diagram  Latency=0  AutoFrameSizeCalculation=off
      link override Signal_Limit/_maxval: Value=KOUTP_HBeam_flg_maxval
      link override Signal_Limit/_minval: Value=KOUTP_HBeam_flg_minval
      link override Signal_Override/_ovrdflg: Value=KOUTP_HBeam_flg_ovrdflg
      link override Signal_Override/_ovrdval: Value=KOUTP_HBeam_flg_ovrdval
  VBCM_HMIKey1FuncSta_enum_Inproc : FVT_lib/outp/OverrideAndLimit  SystemSampleTime=-1  VariantActivationTime=update diagram  Latency=0  AutoFrameSizeCalculation=off
      link override Signal_Limit/_maxval: Value=KOUTP_HMIKey1FuncSta_enum_maxval
      link override Signal_Limit/_minval: Value=KOUTP_HMIKey1FuncSta_enum_minval
      link override Signal_Override/_ovrdflg: Value=KOUTP_HMIKey1FuncSta_enum_ovrdflg
      link override Signal_Override/_ovrdval: Value=KOUTP_HMIKey1FuncSta_enum_ovrdval
  VBCM_HMIKey2FuncSta_enum_Inproc : FVT_lib/outp/OverrideAndLimit  SystemSampleTime=-1  VariantActivationTime=update diagram  Latency=0  AutoFrameSizeCalculation=off
      link override Signal_Limit/_maxval: Value=KOUTP_HMIKey2FuncSta_enum_maxval
      link override Signal_Limit/_minval: Value=KOUTP_HMIKey2FuncSta_enum_minval
      link override Signal_Override/_ovrdflg: Value=KOUTP_HMIKey2FuncSta_enum_ovrdflg
      link override Signal_Override/_ovrdval: Value=KOUTP_HMIKey2FuncSta_enum_ovrdval
  VBCM_HMIKey3FuncSta_enum_Inproc : FVT_lib/outp/OverrideAndLimit  SystemSampleTime=-1  VariantActivationTime=update diagram  Latency=0  AutoFrameSizeCalculation=off
      link override Signal_Limit/_maxval: Value=KOUTP_HMIKey3FuncSta_enum_maxval
      link override Signal_Limit/_minval: Value=KOUTP_HMIKey3FuncSta_enum_minval
      link override Signal_Override/_ovrdflg: Value=KOUTP_HMIKey3FuncSta_enum_ovrdflg
      link override Signal_Override/_ovrdval: Value=KOUTP_HMIKey3FuncSta_enum_ovrdval
  VBCM_HMIKey4FuncSta_enum_Inproc : FVT_lib/outp/OverrideAndLimit  SystemSampleTime=-1  VariantActivationTime=update diagram  Latency=0  AutoFrameSizeCalculation=off
      link override Signal_Limit/_maxval: Value=KOUTP_HMIKey4FuncSta_enum_maxval
      link override Signal_Limit/_minval: Value=KOUTP_HMIKey4FuncSta_enum_minval
      link override Signal_Override/_ovrdflg: Value=KOUTP_HMIKey4FuncSta_enum_ovrdflg
      link override Signal_Override/_ovrdval: Value=KOUTP_HMIKey4FuncSta_enum_ovrdval
  VBCM_HMIKey5FuncSta_enum_Inproc : FVT_lib/outp/OverrideAndLimit  SystemSampleTime=-1  VariantActivationTime=update diagram  Latency=0  AutoFrameSizeCalculation=off
      link override Signal_Limit/_maxval: Value=KOUTP_HMIKey5FuncSta_enum_maxval
      link override Signal_Limit/_minval: Value=KOUTP_HMIKey5FuncSta_enum_minval
      link override Signal_Override/_ovrdflg: Value=KOUTP_HMIKey5FuncSta_enum_ovrdflg
      link override Signal_Override/_ovrdval: Value=KOUTP_HMIKey5FuncSta_enum_ovrdval
  VBCM_HMIKey6FuncSta_enum_Inproc : FVT_lib/outp/OverrideAndLimit  SystemSampleTime=-1  VariantActivationTime=update diagram  Latency=0  AutoFrameSizeCalculation=off
      link override Signal_Limit/_maxval: Value=KOUTP_HMIKey6FuncSta_enum_maxval
      link override Signal_Limit/_minval: Value=KOUTP_HMIKey6FuncSta_enum_minval
      link override Signal_Override/_ovrdflg: Value=KOUTP_HMIKey6FuncSta_enum_ovrdflg
      link override Signal_Override/_ovrdval: Value=KOUTP_HMIKey6FuncSta_enum_ovrdval
  VBCM_HMIKey7FuncSta_enum_Inproc : FVT_lib/outp/OverrideAndLimit  SystemSampleTime=-1  VariantActivationTime=update diagram  Latency=0  AutoFrameSizeCalculation=off
      link override Signal_Limit/_maxval: Value=KOUTP_HMIKey7FuncSta_enum_maxval
      link override Signal_Limit/_minval: Value=KOUTP_HMIKey7FuncSta_enum_minval
      link override Signal_Override/_ovrdflg: Value=KOUTP_HMIKey7FuncSta_enum_ovrdflg
      link override Signal_Override/_ovrdval: Value=KOUTP_HMIKey7FuncSta_enum_ovrdval
  VBCM_HMIKey8FuncSta_enum_Inproc : FVT_lib/outp/OverrideAndLimit  SystemSampleTime=-1  VariantActivationTime=update diagram  Latency=0  AutoFrameSizeCalculation=off
      link override Signal_Limit/_maxval: Value=KOUTP_HMIKey8FuncSta_enum_maxval
      link override Signal_Limit/_minval: Value=KOUTP_HMIKey8FuncSta_enum_minval
      link override Signal_Override/_ovrdflg: Value=KOUTP_HMIKey8FuncSta_enum_ovrdflg
      link override Signal_Override/_ovrdval: Value=KOUTP_HMIKey8FuncSta_enum_ovrdval
  VBCM_HazardIND_flg_Inproc : FVT_lib/outp/OverrideAndLimit  SystemSampleTime=-1  VariantActivationTime=update diagram  Latency=0  AutoFrameSizeCalculation=off
      link override Signal_Limit/_maxval: Value=KOUTP_HazardIND_flg_maxval
      link override Signal_Limit/_minval: Value=KOUTP_HazardIND_flg_minval
      link override Signal_Override/_ovrdflg: Value=KOUTP_HazardIND_flg_ovrdflg
      link override Signal_Override/_ovrdval: Value=KOUTP_HazardIND_flg_ovrdval
  VBCM_HazardSW_flg_Inproc : FVT_lib/outp/OverrideAndLimit  SystemSampleTime=-1  VariantActivationTime=update diagram  Latency=0  AutoFrameSizeCalculation=off
      link override Signal_Limit/_maxval: Value=KOUTP_HazardSW_flg_maxval
      link override Signal_Limit/_minval: Value=KOUTP_HazardSW_flg_minval
      link override Signal_Override/_ovrdflg: Value=KOUTP_HazardSW_flg_ovrdflg
      link override Signal_Override/_ovrdval: Value=KOUTP_HazardSW_flg_ovrdval
  VBCM_HoodRelCmd_flg_Inproc : FVT_lib/outp/OverrideAndLimit  SystemSampleTime=-1  VariantActivationTime=update diagram  Latency=0  AutoFrameSizeCalculation=off
      link override Signal_Limit/_maxval: Value=KOUTP_HoodRelCmd_flg_maxval
      link override Signal_Limit/_minval: Value=KOUTP_HoodRelCmd_flg_minval
      link override Signal_Override/_ovrdflg: Value=KOUTP_HoodRelCmd_flg_ovrdflg
      link override Signal_Override/_ovrdval: Value=KOUTP_HoodRelCmd_flg_ovrdval
  VBCM_HoodSW_flg_Inproc : FVT_lib/outp/OverrideAndLimit  SystemSampleTime=-1  VariantActivationTime=update diagram  Latency=0  AutoFrameSizeCalculation=off
      link override Signal_Limit/_maxval: Value=KOUTP_HoodSW_flg_maxval
      link override Signal_Limit/_minval: Value=KOUTP_HoodSW_flg_minval
      link override Signal_Override/_ovrdflg: Value=KOUTP_HoodSW_flg_ovrdflg
      link override Signal_Override/_ovrdval: Value=KOUTP_HoodSW_flg_ovrdval
  VBCM_HornCtrl_flg_Inproc : FVT_lib/outp/OverrideAndLimit  SystemSampleTime=-1  VariantActivationTime=update diagram  Latency=0  AutoFrameSizeCalculation=off
      link override Signal_Limit/_maxval: Value=KOUTP_HornCtrl_flg_maxval
      link override Signal_Limit/_minval: Value=KOUTP_HornCtrl_flg_minval
      link override Signal_Override/_ovrdflg: Value=KOUTP_HornCtrl_flg_ovrdflg
      link override Signal_Override/_ovrdval: Value=KOUTP_HornCtrl_flg_ovrdval
  VBCM_IVIRST_flg_Inproc : FVT_lib/outp/OverrideAndLimit  SystemSampleTime=-1  VariantActivationTime=update diagram  Latency=0  AutoFrameSizeCalculation=off
      link override Signal_Limit/_maxval: Value=KOUTP_IVIRST_flg_maxval
      link override Signal_Limit/_minval: Value=KOUTP_IVIRST_flg_minval
      link override Signal_Override/_ovrdflg: Value=KOUTP_IVIRST_flg_ovrdflg
      link override Signal_Override/_ovrdval: Value=KOUTP_IVIRST_flg_ovrdval
  VBCM_LBSD_flg_Inproc : FVT_lib/outp/OverrideAndLimit  SystemSampleTime=-1  VariantActivationTime=update diagram  Latency=0  AutoFrameSizeCalculation=off
      link override Signal_Limit/_maxval: Value=KOUTP_LBSD_flg_maxval
      link override Signal_Limit/_minval: Value=KOUTP_LBSD_flg_minval
      link override Signal_Override/_ovrdflg: Value=KOUTP_LBSD_flg_ovrdflg
      link override Signal_Override/_ovrdval: Value=KOUTP_LBSD_flg_ovrdval
  VBCM_LBeam_flg_Inproc : FVT_lib/outp/OverrideAndLimit  SystemSampleTime=-1  VariantActivationTime=update diagram  Latency=0  AutoFrameSizeCalculation=off
      link override Signal_Limit/_maxval: Value=KOUTP_LBeam_flg_maxval
      link override Signal_Limit/_minval: Value=KOUTP_LBeam_flg_minval
      link override Signal_Override/_ovrdflg: Value=KOUTP_LBeam_flg_ovrdflg
      link override Signal_Override/_ovrdval: Value=KOUTP_LBeam_flg_ovrdval
  VBCM_LDRL_flg_Inproc : FVT_lib/outp/OverrideAndLimit  SystemSampleTime=-1  VariantActivationTime=update diagram  Latency=0  AutoFrameSizeCalculation=off
      link override Signal_Limit/_maxval: Value=KOUTP_LDRL_flg_maxval
      link override Signal_Limit/_minval: Value=KOUTP_LDRL_flg_minval
      link override Signal_Override/_ovrdflg: Value=KOUTP_LDRL_flg_ovrdflg
      link override Signal_Override/_ovrdval: Value=KOUTP_LDRL_flg_ovrdval
  VBCM_LLeftStaCmd_flg_Inproc : FVT_lib/outp/OverrideAndLimit  SystemSampleTime=-1  VariantActivationTime=update diagram  Latency=0  AutoFrameSizeCalculation=off
      link override Signal_Limit/_maxval: Value=KOUTP_LLeftStaCmd_flg_maxval
      link override Signal_Limit/_minval: Value=KOUTP_LLeftStaCmd_flg_minval
      link override Signal_Override/_ovrdflg: Value=KOUTP_LLeftStaCmd_flg_ovrdflg
      link override Signal_Override/_ovrdval: Value=KOUTP_LLeftStaCmd_flg_ovrdval
  VBCM_LRightStaCmd_flg_Inproc : FVT_lib/outp/OverrideAndLimit  SystemSampleTime=-1  VariantActivationTime=update diagram  Latency=0  AutoFrameSizeCalculation=off
      link override Signal_Limit/_maxval: Value=KOUTP_LRightStaCmd_flg_maxval
      link override Signal_Limit/_minval: Value=KOUTP_LRightStaCmd_flg_minval
      link override Signal_Override/_ovrdflg: Value=KOUTP_LRightStaCmd_flg_ovrdflg
      link override Signal_Override/_ovrdval: Value=KOUTP_LRightStaCmd_flg_ovrdval
  VBCM_LTurnLP_flg_Inproc : FVT_lib/outp/OverrideAndLimit  SystemSampleTime=-1  VariantActivationTime=update diagram  Latency=0  AutoFrameSizeCalculation=off
      link override Signal_Limit/_maxval: Value=KOUTP_LTurnLP_flg_maxval
      link override Signal_Limit/_minval: Value=KOUTP_LTurnLP_flg_minval
      link override Signal_Override/_ovrdflg: Value=KOUTP_LTurnLP_flg_ovrdflg
      link override Signal_Override/_ovrdval: Value=KOUTP_LTurnLP_flg_ovrdval
  VBCM_LampPwr_flg_Inproc : FVT_lib/outp/OverrideAndLimit  SystemSampleTime=-1  VariantActivationTime=update diagram  Latency=0  AutoFrameSizeCalculation=off
      link override Signal_Limit/_maxval: Value=KOUTP_LampPwr_flg_maxval
      link override Signal_Limit/_minval: Value=KOUTP_LampPwr_flg_minval
      link override Signal_Override/_ovrdflg: Value=KOUTP_LampPwr_flg_ovrdflg
      link override Signal_Override/_ovrdval: Value=KOUTP_LampPwr_flg_ovrdval
  VBCM_LockAlarm_enum_Inproc : FVT_lib/outp/OverrideAndLimit  SystemSampleTime=-1  VariantActivationTime=update diagram  Latency=0  AutoFrameSizeCalculation=off
      link override Signal_Limit/_maxval: Value=KOUTP_LockAlarm_enum_maxval
      link override Signal_Limit/_minval: Value=KOUTP_LockAlarm_enum_minval
      link override Signal_Override/_ovrdflg: Value=KOUTP_LockAlarm_enum_ovrdflg
      link override Signal_Override/_ovrdval: Value=KOUTP_LockAlarm_enum_ovrdval
  VBCM_LockSettingStaMem_enum_Inproc : FVT_lib/outp/OverrideAndLimit  SystemSampleTime=-1  VariantActivationTime=update diagram  Latency=0  AutoFrameSizeCalculation=off
      link override Signal_Limit/_maxval: Value=KOUTP_LockSettingStaMem_enum_maxval
      link override Signal_Limit/_minval: Value=KOUTP_LockSettingStaMem_enum_minval
      link override Signal_Override/_ovrdflg: Value=KOUTP_LockSettingStaMem_enum_ovrdflg
      link override Signal_Override/_ovrdval: Value=KOUTP_LockSettingStaMem_enum_ovrdval
  VBCM_LockSetting_flg_Inproc : FVT_lib/outp/OverrideAndLimit  SystemSampleTime=-1  VariantActivationTime=update diagram  Latency=0  AutoFrameSizeCalculation=off
      link override Signal_Limit/_maxval: Value=KOUTP_LockSetting_flg_maxval
      link override Signal_Limit/_minval: Value=KOUTP_LockSetting_flg_minval
      link override Signal_Override/_ovrdflg: Value=KOUTP_LockSetting_flg_ovrdflg
      link override Signal_Override/_ovrdval: Value=KOUTP_LockSetting_flg_ovrdval
  VBCM_MFRDNBrightReq_pct_Inproc : FVT_lib/outp/OverrideAndLimit  SystemSampleTime=-1  VariantActivationTime=update diagram  Latency=0  AutoFrameSizeCalculation=off
      link override Signal_Limit/_maxval: Value=KOUTP_MFRDNBrightReq_pct_maxval
      link override Signal_Limit/_minval: Value=KOUTP_MFRDNBrightReq_pct_minval
      link override Signal_Override/_ovrdflg: Value=KOUTP_MFRDNBrightReq_pct_ovrdflg
      link override Signal_Override/_ovrdval: Value=KOUTP_MFRDNBrightReq_pct_ovrdval
  VBCM_MFSWTri_flg_Inproc : FVT_lib/outp/OverrideAndLimit  SystemSampleTime=-1  VariantActivationTime=update diagram  Latency=0  AutoFrameSizeCalculation=off
      link override Signal_Limit/_maxval: Value=KOUTP_MFSWTri_flg_maxval
      link override Signal_Limit/_minval: Value=KOUTP_MFSWTri_flg_minval
      link override Signal_Override/_ovrdflg: Value=KOUTP_MFSWTri_flg_ovrdflg
      link override Signal_Override/_ovrdval: Value=KOUTP_MFSWTri_flg_ovrdval
  VBCM_MirrorCtrl_enum_Inproc : FVT_lib/outp/OverrideAndLimit  SystemSampleTime=-1  VariantActivationTime=update diagram  Latency=0  AutoFrameSizeCalculation=off
      link override Signal_Limit/_maxval: Value=KOUTP_MirrorCtrl_enum_maxval
      link override Signal_Limit/_minval: Value=KOUTP_MirrorCtrl_enum_minval
      link override Signal_Override/_ovrdflg: Value=KOUTP_MirrorCtrl_enum_ovrdflg
      link override Signal_Override/_ovrdval: Value=KOUTP_MirrorCtrl_enum_ovrdval
  VBCM_MirrorDefog_flg_Inproc : FVT_lib/outp/OverrideAndLimit  SystemSampleTime=-1  VariantActivationTime=update diagram  Latency=0  AutoFrameSizeCalculation=off
      link override Signal_Limit/_maxval: Value=KOUTP_MirrorDefog_flg_maxval
      link override Signal_Limit/_minval: Value=KOUTP_MirrorDefog_flg_minval
      link override Signal_Override/_ovrdflg: Value=KOUTP_MirrorDefog_flg_ovrdflg
      link override Signal_Override/_ovrdval: Value=KOUTP_MirrorDefog_flg_ovrdval
  VBCM_MirrorFlodPos_flg_Inproc : FVT_lib/outp/OverrideAndLimit  SystemSampleTime=-1  VariantActivationTime=update diagram  Latency=0  AutoFrameSizeCalculation=off
      link override Signal_Limit/_maxval: Value=KOUTP_MirrorFlodPos_flg_maxval
      link override Signal_Limit/_minval: Value=KOUTP_MirrorFlodPos_flg_minval
      link override Signal_Override/_ovrdflg: Value=KOUTP_MirrorFlodPos_flg_ovrdflg
      link override Signal_Override/_ovrdval: Value=KOUTP_MirrorFlodPos_flg_ovrdval
  VBCM_OutMode_enum_Inproc : FVT_lib/outp/OverrideAndLimit  SystemSampleTime=-1  VariantActivationTime=update diagram  Latency=0  AutoFrameSizeCalculation=off
      link override Signal_Limit/_maxval: Value=KOUTP_OutMode_enum_maxval
      link override Signal_Limit/_minval: Value=KOUTP_OutMode_enum_minval
      link override Signal_Override/_ovrdflg: Value=KOUTP_OutMode_enum_ovrdflg
      link override Signal_Override/_ovrdval: Value=KOUTP_OutMode_enum_ovrdval
  VBCM_PTGInnerSW2_enum_Inproc : FVT_lib/outp/OverrideAndLimit  SystemSampleTime=-1  VariantActivationTime=update diagram  Latency=0  AutoFrameSizeCalculation=off
      link override Signal_Limit/_maxval: Value=KOUTP_PTGInnerSW2_enum_maxval
      link override Signal_Limit/_minval: Value=KOUTP_PTGInnerSW2_enum_minval
      link override Signal_Override/_ovrdflg: Value=KOUTP_PTGInnerSW2_enum_ovrdflg
      link override Signal_Override/_ovrdval: Value=KOUTP_PTGInnerSW2_enum_ovrdval
  VBCM_PTGOpenHeight12_enum_Inproc : FVT_lib/outp/OverrideAndLimit  SystemSampleTime=-1  VariantActivationTime=update diagram  Latency=0  AutoFrameSizeCalculation=off
      link override Signal_Limit/_maxval: Value=KOUTP_PTGOpenHeight12_enum_maxval
      link override Signal_Limit/_minval: Value=KOUTP_PTGOpenHeight12_enum_minval
      link override Signal_Override/_ovrdflg: Value=KOUTP_PTGOpenHeight12_enum_ovrdflg
      link override Signal_Override/_ovrdval: Value=KOUTP_PTGOpenHeight12_enum_ovrdval
  VBCM_PTGOpenHeight34_enum_Inproc : FVT_lib/outp/OverrideAndLimit  SystemSampleTime=-1  VariantActivationTime=update diagram  Latency=0  AutoFrameSizeCalculation=off
      link override Signal_Limit/_maxval: Value=KOUTP_PTGOpenHeight34_enum_maxval
      link override Signal_Limit/_minval: Value=KOUTP_PTGOpenHeight34_enum_minval
      link override Signal_Override/_ovrdflg: Value=KOUTP_PTGOpenHeight34_enum_ovrdflg
      link override Signal_Override/_ovrdval: Value=KOUTP_PTGOpenHeight34_enum_ovrdval
  VBCM_PTGOpenHeight57_enum_Inproc : FVT_lib/outp/OverrideAndLimit  SystemSampleTime=-1  VariantActivationTime=update diagram  Latency=0  AutoFrameSizeCalculation=off
      link override Signal_Limit/_maxval: Value=KOUTP_PTGOpenHeight57_enum_maxval
      link override Signal_Limit/_minval: Value=KOUTP_PTGOpenHeight57_enum_minval
      link override Signal_Override/_ovrdflg: Value=KOUTP_PTGOpenHeight57_enum_ovrdflg
      link override Signal_Override/_ovrdval: Value=KOUTP_PTGOpenHeight57_enum_ovrdval
  VBCM_PTGOpenHeightSta_enum_Inproc : FVT_lib/outp/OverrideAndLimit  SystemSampleTime=-1  VariantActivationTime=update diagram  Latency=0  AutoFrameSizeCalculation=off
      link override Signal_Limit/_maxval: Value=KOUTP_PTGOpenHeightSta_enum_maxval
      link override Signal_Limit/_minval: Value=KOUTP_PTGOpenHeightSta_enum_minval
      link override Signal_Override/_ovrdflg: Value=KOUTP_PTGOpenHeightSta_enum_ovrdflg
      link override Signal_Override/_ovrdval: Value=KOUTP_PTGOpenHeightSta_enum_ovrdval
  VBCM_PTGUserHeight1_cnt_Inproc : FVT_lib/outp/OverrideAndLimit  SystemSampleTime=-1  VariantActivationTime=update diagram  Latency=0  AutoFrameSizeCalculation=off
      link override Signal_Limit/_maxval: Value=KOUTP_PTGUserHeight1_cnt_maxval
      link override Signal_Limit/_minval: Value=KOUTP_PTGUserHeight1_cnt_minval
      link override Signal_Override/_ovrdflg: Value=KOUTP_PTGUserHeight1_cnt_ovrdflg
      link override Signal_Override/_ovrdval: Value=KOUTP_PTGUserHeight1_cnt_ovrdval
  VBCM_PTGUserHeight2_cnt_Inproc : FVT_lib/outp/OverrideAndLimit  SystemSampleTime=-1  VariantActivationTime=update diagram  Latency=0  AutoFrameSizeCalculation=off
      link override Signal_Limit/_maxval: Value=KOUTP_PTGUserHeight2_cnt_maxval
      link override Signal_Limit/_minval: Value=KOUTP_PTGUserHeight2_cnt_minval
      link override Signal_Override/_ovrdflg: Value=KOUTP_PTGUserHeight2_cnt_ovrdflg
      link override Signal_Override/_ovrdval: Value=KOUTP_PTGUserHeight2_cnt_ovrdval
  VBCM_PTGUserHeight3_cnt_Inproc : FVT_lib/outp/OverrideAndLimit  SystemSampleTime=-1  VariantActivationTime=update diagram  Latency=0  AutoFrameSizeCalculation=off
      link override Signal_Limit/_maxval: Value=KOUTP_PTGUserHeight3_cnt_maxval
      link override Signal_Limit/_minval: Value=KOUTP_PTGUserHeight3_cnt_minval
      link override Signal_Override/_ovrdflg: Value=KOUTP_PTGUserHeight3_cnt_ovrdflg
      link override Signal_Override/_ovrdval: Value=KOUTP_PTGUserHeight3_cnt_ovrdval
  VBCM_PTGUserHeight4_cnt_Inproc : FVT_lib/outp/OverrideAndLimit  SystemSampleTime=-1  VariantActivationTime=update diagram  Latency=0  AutoFrameSizeCalculation=off
      link override Signal_Limit/_maxval: Value=KOUTP_PTGUserHeight4_cnt_maxval
      link override Signal_Limit/_minval: Value=KOUTP_PTGUserHeight4_cnt_minval
      link override Signal_Override/_ovrdflg: Value=KOUTP_PTGUserHeight4_cnt_ovrdflg
      link override Signal_Override/_ovrdval: Value=KOUTP_PTGUserHeight4_cnt_ovrdval
  VBCM_PTGUserHeight5_cnt_Inproc : FVT_lib/outp/OverrideAndLimit  SystemSampleTime=-1  VariantActivationTime=update diagram  Latency=0  AutoFrameSizeCalculation=off
      link override Signal_Limit/_maxval: Value=KOUTP_PTGUserHeight5_cnt_maxval
      link override Signal_Limit/_minval: Value=KOUTP_PTGUserHeight5_cnt_minval
      link override Signal_Override/_ovrdflg: Value=KOUTP_PTGUserHeight5_cnt_ovrdflg
      link override Signal_Override/_ovrdval: Value=KOUTP_PTGUserHeight5_cnt_ovrdval
  VBCM_PTGUserHeight7_cnt_Inproc : FVT_lib/outp/OverrideAndLimit  SystemSampleTime=-1  VariantActivationTime=update diagram  Latency=0  AutoFrameSizeCalculation=off
      link override Signal_Limit/_maxval: Value=KOUTP_PTGUserHeight7_cnt_maxval
      link override Signal_Limit/_minval: Value=KOUTP_PTGUserHeight7_cnt_minval
      link override Signal_Override/_ovrdflg: Value=KOUTP_PTGUserHeight7_cnt_ovrdflg
      link override Signal_Override/_ovrdval: Value=KOUTP_PTGUserHeight7_cnt_ovrdval
  VBCM_PasWdwCtrlCmd_pct_Inproc : FVT_lib/outp/OverrideAndLimit  SystemSampleTime=-1  VariantActivationTime=update diagram  Latency=0  AutoFrameSizeCalculation=off
      link override Signal_Limit/_maxval: Value=KOUTP_PasWdwCtrlCmd_pct_maxval
      link override Signal_Limit/_minval: Value=KOUTP_PasWdwCtrlCmd_pct_minval
      link override Signal_Override/_ovrdflg: Value=KOUTP_PasWdwCtrlCmd_pct_ovrdflg
      link override Signal_Override/_ovrdval: Value=KOUTP_PasWdwCtrlCmd_pct_ovrdval
  VBCM_PasWdwReqAP_enum_Inproc : FVT_lib/outp/OverrideAndLimit  SystemSampleTime=-1  VariantActivationTime=update diagram  Latency=0  AutoFrameSizeCalculation=off
      link override Signal_Limit/_maxval: Value=KOUTP_PasWdwReqAP_enum_maxval
      link override Signal_Limit/_minval: Value=KOUTP_PasWdwReqAP_enum_minval
      link override Signal_Override/_ovrdflg: Value=KOUTP_PasWdwReqAP_enum_ovrdflg
      link override Signal_Override/_ovrdval: Value=KOUTP_PasWdwReqAP_enum_ovrdval
  VBCM_PassSWSta_flg_Inproc : FVT_lib/outp/OverrideAndLimit  SystemSampleTime=-1  VariantActivationTime=update diagram  Latency=0  AutoFrameSizeCalculation=off
      link override Signal_Limit/_maxval: Value=KOUTP_PassSWSta_flg_maxval
      link override Signal_Limit/_minval: Value=KOUTP_PassSWSta_flg_minval
      link override Signal_Override/_ovrdflg: Value=KOUTP_PassSWSta_flg_ovrdflg
      link override Signal_Override/_ovrdval: Value=KOUTP_PassSWSta_flg_ovrdval
  VBCM_PosLamp_flg_Inproc : FVT_lib/outp/OverrideAndLimit  SystemSampleTime=-1  VariantActivationTime=update diagram  Latency=0  AutoFrameSizeCalculation=off
      link override Signal_Limit/_maxval: Value=KOUTP_PosLamp_flg_maxval
      link override Signal_Limit/_minval: Value=KOUTP_PosLamp_flg_minval
      link override Signal_Override/_ovrdflg: Value=KOUTP_PosLamp_flg_ovrdflg
      link override Signal_Override/_ovrdval: Value=KOUTP_PosLamp_flg_ovrdval
  VBCM_PsDoorSW_flg_Inproc : FVT_lib/outp/OverrideAndLimit  SystemSampleTime=-1  VariantActivationTime=update diagram  Latency=0  AutoFrameSizeCalculation=off
      link override Signal_Limit/_maxval: Value=KOUTP_PsDoorSW_flg_maxval
      link override Signal_Limit/_minval: Value=KOUTP_PsDoorSW_flg_minval
      link override Signal_Override/_ovrdflg: Value=KOUTP_PsDoorSW_flg_ovrdflg
      link override Signal_Override/_ovrdval: Value=KOUTP_PsDoorSW_flg_ovrdval
  VBCM_PsRWdwCtrlCmd_pct_Inproc : FVT_lib/outp/OverrideAndLimit  SystemSampleTime=-1  VariantActivationTime=update diagram  Latency=0  AutoFrameSizeCalculation=off
      link override Signal_Limit/_maxval: Value=KOUTP_PsRWdwCtrlCmd_pct_maxval
      link override Signal_Limit/_minval: Value=KOUTP_PsRWdwCtrlCmd_pct_minval
      link override Signal_Override/_ovrdflg: Value=KOUTP_PsRWdwCtrlCmd_pct_ovrdflg
      link override Signal_Override/_ovrdval: Value=KOUTP_PsRWdwCtrlCmd_pct_ovrdval
  VBCM_PsRWdwReqAP_enum_Inproc : FVT_lib/outp/OverrideAndLimit  SystemSampleTime=-1  VariantActivationTime=update diagram  Latency=0  AutoFrameSizeCalculation=off
      link override Signal_Limit/_maxval: Value=KOUTP_PsRWdwReqAP_enum_maxval
      link override Signal_Limit/_minval: Value=KOUTP_PsRWdwReqAP_enum_minval
      link override Signal_Override/_ovrdflg: Value=KOUTP_PsRWdwReqAP_enum_ovrdflg
      link override Signal_Override/_ovrdval: Value=KOUTP_PsRWdwReqAP_enum_ovrdval
  VBCM_RBSD_flg_Inproc : FVT_lib/outp/OverrideAndLimit  SystemSampleTime=-1  VariantActivationTime=update diagram  Latency=0  AutoFrameSizeCalculation=off
      link override Signal_Limit/_maxval: Value=KOUTP_RBSD_flg_maxval
      link override Signal_Limit/_minval: Value=KOUTP_RBSD_flg_minval
      link override Signal_Override/_ovrdflg: Value=KOUTP_RBSD_flg_ovrdflg
      link override Signal_Override/_ovrdval: Value=KOUTP_RBSD_flg_ovrdval
  VBCM_RDRL_flg_Inproc : FVT_lib/outp/OverrideAndLimit  SystemSampleTime=-1  VariantActivationTime=update diagram  Latency=0  AutoFrameSizeCalculation=off
      link override Signal_Limit/_maxval: Value=KOUTP_RDRL_flg_maxval
      link override Signal_Limit/_minval: Value=KOUTP_RDRL_flg_minval
      link override Signal_Override/_ovrdflg: Value=KOUTP_RDRL_flg_ovrdflg
      link override Signal_Override/_ovrdval: Value=KOUTP_RDRL_flg_ovrdval
  VBCM_RLDoorSW_flg_Inproc : FVT_lib/outp/OverrideAndLimit  SystemSampleTime=-1  VariantActivationTime=update diagram  Latency=0  AutoFrameSizeCalculation=off
      link override Signal_Limit/_maxval: Value=KOUTP_RLDoorSW_flg_maxval
      link override Signal_Limit/_minval: Value=KOUTP_RLDoorSW_flg_minval
      link override Signal_Override/_ovrdflg: Value=KOUTP_RLDoorSW_flg_ovrdflg
      link override Signal_Override/_ovrdval: Value=KOUTP_RLDoorSW_flg_ovrdval
  VBCM_RRDoorSW_flg_Inproc : FVT_lib/outp/OverrideAndLimit  SystemSampleTime=-1  VariantActivationTime=update diagram  Latency=0  AutoFrameSizeCalculation=off
      link override Signal_Limit/_maxval: Value=KOUTP_RRDoorSW_flg_maxval
      link override Signal_Limit/_minval: Value=KOUTP_RRDoorSW_flg_minval
      link override Signal_Override/_ovrdflg: Value=KOUTP_RRDoorSW_flg_ovrdflg
      link override Signal_Override/_ovrdval: Value=KOUTP_RRDoorSW_flg_ovrdval
  VBCM_RTurnLP_flg_Inproc : FVT_lib/outp/OverrideAndLimit  SystemSampleTime=-1  VariantActivationTime=update diagram  Latency=0  AutoFrameSizeCalculation=off
      link override Signal_Limit/_maxval: Value=KOUTP_RTurnLP_flg_maxval
      link override Signal_Limit/_minval: Value=KOUTP_RTurnLP_flg_minval
      link override Signal_Override/_ovrdflg: Value=KOUTP_RTurnLP_flg_ovrdflg
      link override Signal_Override/_ovrdval: Value=KOUTP_RTurnLP_flg_ovrdval
  VBCM_ReverseLamp_flg_Inproc : FVT_lib/outp/OverrideAndLimit  SystemSampleTime=-1  VariantActivationTime=update diagram  Latency=0  AutoFrameSizeCalculation=off
      link override Signal_Limit/_maxval: Value=KOUTP_ReverseLamp_flg_maxval
      link override Signal_Limit/_minval: Value=KOUTP_ReverseLamp_flg_minval
      link override Signal_Override/_ovrdflg: Value=KOUTP_ReverseLamp_flg_ovrdflg
      link override Signal_Override/_ovrdval: Value=KOUTP_ReverseLamp_flg_ovrdval
  VBCM_RmLpModeENFunSta_flg_Inproc : FVT_lib/outp/OverrideAndLimit  SystemSampleTime=-1  VariantActivationTime=update diagram  Latency=0  AutoFrameSizeCalculation=off
      link override Signal_Limit/_maxval: Value=KOUTP_RmLpModeENFunSta_flg_maxval
      link override Signal_Limit/_minval: Value=KOUTP_RmLpModeENFunSta_flg_minval
      link override Signal_Override/_ovrdflg: Value=KOUTP_RmLpModeENFunSta_flg_ovrdflg
      link override Signal_Override/_ovrdval: Value=KOUTP_RmLpModeENFunSta_flg_ovrdval
  VBCM_RmLpModeENMem_enum_Inproc : FVT_lib/outp/OverrideAndLimit  SystemSampleTime=-1  VariantActivationTime=update diagram  Latency=0  AutoFrameSizeCalculation=off
      link override Signal_Limit/_maxval: Value=KOUTP_RmLpModeENMem_enum_maxval
      link override Signal_Limit/_minval: Value=KOUTP_RmLpModeENMem_enum_minval
      link override Signal_Override/_ovrdflg: Value=KOUTP_RmLpModeENMem_enum_ovrdflg
      link override Signal_Override/_ovrdval: Value=KOUTP_RmLpModeENMem_enum_ovrdval
  VBCM_RoomLampH_flg_Inproc : FVT_lib/outp/OverrideAndLimit  SystemSampleTime=-1  VariantActivationTime=update diagram  Latency=0  AutoFrameSizeCalculation=off
      link override Signal_Limit/_maxval: Value=KOUTP_RoomLampH_flg_maxval
      link override Signal_Limit/_minval: Value=KOUTP_RoomLampH_flg_minval
      link override Signal_Override/_ovrdflg: Value=KOUTP_RoomLampH_flg_ovrdflg
      link override Signal_Override/_ovrdval: Value=KOUTP_RoomLampH_flg_ovrdval
  VBCM_RoomLampL_flg_Inproc : FVT_lib/outp/OverrideAndLimit  SystemSampleTime=-1  VariantActivationTime=update diagram  Latency=0  AutoFrameSizeCalculation=off
      link override Signal_Limit/_maxval: Value=KOUTP_RoomLampL_flg_maxval
      link override Signal_Limit/_minval: Value=KOUTP_RoomLampL_flg_minval
      link override Signal_Override/_ovrdflg: Value=KOUTP_RoomLampL_flg_ovrdflg
      link override Signal_Override/_ovrdval: Value=KOUTP_RoomLampL_flg_ovrdval
  VBCM_RrChargingDoorCtrl_enum_Inproc : FVT_lib/outp/OverrideAndLimit  SystemSampleTime=-1  VariantActivationTime=update diagram  Latency=0  AutoFrameSizeCalculation=off
      link override Signal_Limit/_maxval: Value=KOUTP_RrChargingDoorCtrl_enum_maxval
      link override Signal_Limit/_minval: Value=KOUTP_RrChargingDoorCtrl_enum_minval
      link override Signal_Override/_ovrdflg: Value=KOUTP_RrChargingDoorCtrl_enum_ovrdflg
      link override Signal_Override/_ovrdval: Value=KOUTP_RrChargingDoorCtrl_enum_ovrdval
  VBCM_RrDefog_flg_Inproc : FVT_lib/outp/OverrideAndLimit  SystemSampleTime=-1  VariantActivationTime=update diagram  Latency=0  AutoFrameSizeCalculation=off
      link override Signal_Limit/_maxval: Value=KOUTP_RrDefog_flg_maxval
      link override Signal_Limit/_minval: Value=KOUTP_RrDefog_flg_minval
      link override Signal_Override/_ovrdflg: Value=KOUTP_RrDefog_flg_ovrdflg
      link override Signal_Override/_ovrdval: Value=KOUTP_RrDefog_flg_ovrdval
  VBCM_RrFogLamp_flg_Inproc : FVT_lib/outp/OverrideAndLimit  SystemSampleTime=-1  VariantActivationTime=update diagram  Latency=0  AutoFrameSizeCalculation=off
      link override Signal_Limit/_maxval: Value=KOUTP_RrFogLamp_flg_maxval
      link override Signal_Limit/_minval: Value=KOUTP_RrFogLamp_flg_minval
      link override Signal_Override/_ovrdflg: Value=KOUTP_RrFogLamp_flg_ovrdflg
      link override Signal_Override/_ovrdval: Value=KOUTP_RrFogLamp_flg_ovrdval
  VBCM_RrWiper_flg_Inproc : FVT_lib/outp/OverrideAndLimit  SystemSampleTime=-1  VariantActivationTime=update diagram  Latency=0  AutoFrameSizeCalculation=off
      link override Signal_Limit/_maxval: Value=KOUTP_RrWiper_flg_maxval
      link override Signal_Limit/_minval: Value=KOUTP_RrWiper_flg_minval
      link override Signal_Override/_ovrdflg: Value=KOUTP_RrWiper_flg_ovrdflg
      link override Signal_Override/_ovrdval: Value=KOUTP_RrWiper_flg_ovrdval
  VBCM_SPTGDet_flg_Inproc : FVT_lib/outp/OverrideAndLimit  SystemSampleTime=-1  VariantActivationTime=update diagram  Latency=0  AutoFrameSizeCalculation=off
      link override Signal_Limit/_maxval: Value=KOUTP_SPTGDet_flg_maxval
      link override Signal_Limit/_minval: Value=KOUTP_SPTGDet_flg_minval
      link override Signal_Override/_ovrdflg: Value=KOUTP_SPTGDet_flg_ovrdflg
      link override Signal_Override/_ovrdval: Value=KOUTP_SPTGDet_flg_ovrdval
  VBCM_SPTGENFunMem_enum_Inproc : FVT_lib/outp/OverrideAndLimit  SystemSampleTime=-1  VariantActivationTime=update diagram  Latency=0  AutoFrameSizeCalculation=off
      link override Signal_Limit/_maxval: Value=KOUTP_SPTGENFunMem_enum_maxval
      link override Signal_Limit/_minval: Value=KOUTP_SPTGENFunMem_enum_minval
      link override Signal_Override/_ovrdflg: Value=KOUTP_SPTGENFunMem_enum_ovrdflg
      link override Signal_Override/_ovrdval: Value=KOUTP_SPTGENFunMem_enum_ovrdval
  VBCM_SPTGENFun_flg_Inproc : FVT_lib/outp/OverrideAndLimit  SystemSampleTime=-1  VariantActivationTime=update diagram  Latency=0  AutoFrameSizeCalculation=off
      link override Signal_Limit/_maxval: Value=KOUTP_SPTGENFun_flg_maxval
      link override Signal_Limit/_minval: Value=KOUTP_SPTGENFun_flg_minval
      link override Signal_Override/_ovrdflg: Value=KOUTP_SPTGENFun_flg_ovrdflg
      link override Signal_Override/_ovrdval: Value=KOUTP_SPTGENFun_flg_ovrdval
  VBCM_SenstivityPosnCmd_enum_Inproc : FVT_lib/outp/OverrideAndLimit  SystemSampleTime=-1  VariantActivationTime=update diagram  Latency=0  AutoFrameSizeCalculation=off
      link override Signal_Limit/_maxval: Value=KOUTP_SenstivityPosnCmd_enum_maxval
      link override Signal_Limit/_minval: Value=KOUTP_SenstivityPosnCmd_enum_minval
      link override Signal_Override/_ovrdflg: Value=KOUTP_SenstivityPosnCmd_enum_ovrdflg
      link override Signal_Override/_ovrdval: Value=KOUTP_SenstivityPosnCmd_enum_ovrdval
  VBCM_TailgateHDSW_flg_Inproc : FVT_lib/outp/OverrideAndLimit  SystemSampleTime=-1  VariantActivationTime=update diagram  Latency=0  AutoFrameSizeCalculation=off
      link override Signal_Limit/_maxval: Value=KOUTP_TailgateHDSW_flg_maxval
      link override Signal_Limit/_minval: Value=KOUTP_TailgateHDSW_flg_minval
      link override Signal_Override/_ovrdflg: Value=KOUTP_TailgateHDSW_flg_ovrdflg
      link override Signal_Override/_ovrdval: Value=KOUTP_TailgateHDSW_flg_ovrdval
  VBCM_TailgateRemote_enum_Inproc : FVT_lib/outp/OverrideAndLimit  SystemSampleTime=-1  VariantActivationTime=update diagram  Latency=0  AutoFrameSizeCalculation=off
      link override Signal_Limit/_maxval: Value=KOUTP_TailgateRemote_enum_maxval
      link override Signal_Limit/_minval: Value=KOUTP_TailgateRemote_enum_minval
      link override Signal_Override/_ovrdflg: Value=KOUTP_TailgateRemote_enum_ovrdflg
      link override Signal_Override/_ovrdval: Value=KOUTP_TailgateRemote_enum_ovrdval
  VBCM_TailgateSW_flg_Inproc : FVT_lib/outp/OverrideAndLimit  SystemSampleTime=-1  VariantActivationTime=update diagram  Latency=0  AutoFrameSizeCalculation=off
      link override Signal_Limit/_maxval: Value=KOUTP_TailgateSW_flg_maxval
      link override Signal_Limit/_minval: Value=KOUTP_TailgateSW_flg_minval
      link override Signal_Override/_ovrdflg: Value=KOUTP_TailgateSW_flg_ovrdflg
      link override Signal_Override/_ovrdval: Value=KOUTP_TailgateSW_flg_ovrdval
  VBCM_TimeGapLevelSta_enum_Inproc : FVT_lib/outp/OverrideAndLimit  SystemSampleTime=-1  VariantActivationTime=update diagram  Latency=0  AutoFrameSizeCalculation=off
      link override Signal_Limit/_maxval: Value=KOUTP_TimeGapLevelSta_enum_maxval
      link override Signal_Limit/_minval: Value=KOUTP_TimeGapLevelSta_enum_minval
      link override Signal_Override/_ovrdflg: Value=KOUTP_TimeGapLevelSta_enum_ovrdflg
      link override Signal_Override/_ovrdval: Value=KOUTP_TimeGapLevelSta_enum_ovrdval
  VBCM_TrunkRel_flg_Inproc : FVT_lib/outp/OverrideAndLimit  SystemSampleTime=-1  VariantActivationTime=update diagram  Latency=0  AutoFrameSizeCalculation=off
      link override Signal_Limit/_maxval: Value=KOUTP_TrunkRel_flg_maxval
      link override Signal_Limit/_minval: Value=KOUTP_TrunkRel_flg_minval
      link override Signal_Override/_ovrdflg: Value=KOUTP_TrunkRel_flg_ovrdflg
      link override Signal_Override/_ovrdval: Value=KOUTP_TrunkRel_flg_ovrdval
  VBCM_TurnSwSta_enum_Inproc : FVT_lib/outp/OverrideAndLimit  SystemSampleTime=-1  VariantActivationTime=update diagram  Latency=0  AutoFrameSizeCalculation=off
      link override Signal_Limit/_maxval: Value=KOUTP_TurnSwSta_enum_maxval
      link override Signal_Limit/_minval: Value=KOUTP_TurnSwSta_enum_minval
      link override Signal_Override/_ovrdflg: Value=KOUTP_TurnSwSta_enum_ovrdflg
      link override Signal_Override/_ovrdval: Value=KOUTP_TurnSwSta_enum_ovrdval
  VBCM_TurnSwTSetSta_enum_Inproc : FVT_lib/outp/OverrideAndLimit  SystemSampleTime=-1  VariantActivationTime=update diagram  Latency=0  AutoFrameSizeCalculation=off
      link override Signal_Limit/_maxval: Value=KOUTP_TurnSwTSetSta_enum_maxval
      link override Signal_Limit/_minval: Value=KOUTP_TurnSwTSetSta_enum_minval
      link override Signal_Override/_ovrdflg: Value=KOUTP_TurnSwTSetSta_enum_ovrdflg
      link override Signal_Override/_ovrdval: Value=KOUTP_TurnSwTSetSta_enum_ovrdval
  VBCM_TurnSwTimeSetSta123_enum_Inproc : FVT_lib/outp/OverrideAndLimit  SystemSampleTime=-1  VariantActivationTime=update diagram  Latency=0  AutoFrameSizeCalculation=off
      link override Signal_Limit/_maxval: Value=KOUTP_TurnSwTimeSetSta123_enum_maxval
      link override Signal_Limit/_minval: Value=KOUTP_TurnSwTimeSetSta123_enum_minval
      link override Signal_Override/_ovrdflg: Value=KOUTP_TurnSwTimeSetSta123_enum_ovrdflg
      link override Signal_Override/_ovrdval: Value=KOUTP_TurnSwTimeSetSta123_enum_ovrdval
  VBCM_TurnSwTimeSetSta457_enum_Inproc : FVT_lib/outp/OverrideAndLimit  SystemSampleTime=-1  VariantActivationTime=update diagram  Latency=0  AutoFrameSizeCalculation=off
      link override Signal_Limit/_maxval: Value=KOUTP_TurnSwTimeSetSta457_enum_maxval
      link override Signal_Limit/_minval: Value=KOUTP_TurnSwTimeSetSta457_enum_minval
      link override Signal_Override/_ovrdflg: Value=KOUTP_TurnSwTimeSetSta457_enum_ovrdflg
      link override Signal_Override/_ovrdval: Value=KOUTP_TurnSwTimeSetSta457_enum_ovrdval
  VBCM_UserHeightSet_cnt_Inproc : FVT_lib/outp/OverrideAndLimit  SystemSampleTime=-1  VariantActivationTime=update diagram  Latency=0  AutoFrameSizeCalculation=off
      link override Signal_Limit/_maxval: Value=KOUTP_UserHeightSet_cnt_maxval
      link override Signal_Limit/_minval: Value=KOUTP_UserHeightSet_cnt_minval
      link override Signal_Override/_ovrdflg: Value=KOUTP_UserHeightSet_cnt_ovrdflg
      link override Signal_Override/_ovrdval: Value=KOUTP_UserHeightSet_cnt_ovrdval
  VBCM_UserNow_enum_Inproc : FVT_lib/outp/OverrideAndLimit  SystemSampleTime=-1  VariantActivationTime=update diagram  Latency=0  AutoFrameSizeCalculation=off
      link override Signal_Limit/_maxval: Value=KOUTP_UserNow_enum_maxval
      link override Signal_Limit/_minval: Value=KOUTP_UserNow_enum_minval
      link override Signal_Override/_ovrdflg: Value=KOUTP_UserNow_enum_ovrdflg
      link override Signal_Override/_ovrdval: Value=KOUTP_UserNow_enum_ovrdval
  VBCM_WalkInUnLkENFunSta_flg_Inproc : FVT_lib/outp/OverrideAndLimit  SystemSampleTime=-1  VariantActivationTime=update diagram  Latency=0  AutoFrameSizeCalculation=off
      link override Signal_Limit/_maxval: Value=KOUTP_WalkInUnLkENFunSta_flg_maxval
      link override Signal_Limit/_minval: Value=KOUTP_WalkInUnLkENFunSta_flg_minval
      link override Signal_Override/_ovrdflg: Value=KOUTP_WalkInUnLkENFunSta_flg_ovrdflg
      link override Signal_Override/_ovrdval: Value=KOUTP_WalkInUnLkENFunSta_flg_ovrdval
  VBCM_WalkInUnLkENMem_enum_Inproc : FVT_lib/outp/OverrideAndLimit  SystemSampleTime=-1  VariantActivationTime=update diagram  Latency=0  AutoFrameSizeCalculation=off
      link override Signal_Limit/_maxval: Value=KOUTP_WalkInUnLkENMem_enum_maxval
      link override Signal_Limit/_minval: Value=KOUTP_WalkInUnLkENMem_enum_minval
      link override Signal_Override/_ovrdflg: Value=KOUTP_WalkInUnLkENMem_enum_ovrdflg
      link override Signal_Override/_ovrdval: Value=KOUTP_WalkInUnLkENMem_enum_ovrdval
  VBCM_WalkOutLkENFunSta_flg_Inproc : FVT_lib/outp/OverrideAndLimit  SystemSampleTime=-1  VariantActivationTime=update diagram  Latency=0  AutoFrameSizeCalculation=off
      link override Signal_Limit/_maxval: Value=KOUTP_WalkOutLkENFunSta_flg_maxval
      link override Signal_Limit/_minval: Value=KOUTP_WalkOutLkENFunSta_flg_minval
      link override Signal_Override/_ovrdflg: Value=KOUTP_WalkOutLkENFunSta_flg_ovrdflg
      link override Signal_Override/_ovrdval: Value=KOUTP_WalkOutLkENFunSta_flg_ovrdval
  VBCM_WalkOutLkENMem_enum_Inproc : FVT_lib/outp/OverrideAndLimit  SystemSampleTime=-1  VariantActivationTime=update diagram  Latency=0  AutoFrameSizeCalculation=off
      link override Signal_Limit/_maxval: Value=KOUTP_WalkOutLkENMem_enum_maxval
      link override Signal_Limit/_minval: Value=KOUTP_WalkOutLkENMem_enum_minval
      link override Signal_Override/_ovrdflg: Value=KOUTP_WalkOutLkENMem_enum_ovrdflg
      link override Signal_Override/_ovrdval: Value=KOUTP_WalkOutLkENMem_enum_ovrdval
  VBCM_WasherCtrl_enum_Inproc : FVT_lib/outp/OverrideAndLimit  SystemSampleTime=-1  VariantActivationTime=update diagram  Latency=0  AutoFrameSizeCalculation=off
      link override Signal_Limit/_maxval: Value=KOUTP_WasherCtrl_enum_maxval
      link override Signal_Limit/_minval: Value=KOUTP_WasherCtrl_enum_minval
      link override Signal_Override/_ovrdflg: Value=KOUTP_WasherCtrl_enum_ovrdflg
      link override Signal_Override/_ovrdval: Value=KOUTP_WasherCtrl_enum_ovrdval
  VBCM_WelcomeLight_enum_Inproc : FVT_lib/outp/OverrideAndLimit  SystemSampleTime=-1  VariantActivationTime=update diagram  Latency=0  AutoFrameSizeCalculation=off
      link override Signal_Limit/_maxval: Value=KOUTP_WelcomeLight_enum_maxval
      link override Signal_Limit/_minval: Value=KOUTP_WelcomeLight_enum_minval
      link override Signal_Override/_ovrdflg: Value=KOUTP_WelcomeLight_enum_ovrdflg
      link override Signal_Override/_ovrdval: Value=KOUTP_WelcomeLight_enum_ovrdval
  VBCM_WinLFOpenedSta_pct_Inproc : FVT_lib/outp/OverrideAndLimit  SystemSampleTime=-1  VariantActivationTime=update diagram  Latency=0  AutoFrameSizeCalculation=off
      link override Signal_Limit/_maxval: Value=KOUTP_WinLFOpenedSta_pct_maxval
      link override Signal_Limit/_minval: Value=KOUTP_WinLFOpenedSta_pct_minval
      link override Signal_Override/_ovrdflg: Value=KOUTP_WinLFOpenedSta_pct_ovrdflg
      link override Signal_Override/_ovrdval: Value=KOUTP_WinLFOpenedSta_pct_ovrdval
  VBCM_WinLROpenedSta_pct_Inproc : FVT_lib/outp/OverrideAndLimit  SystemSampleTime=-1  VariantActivationTime=update diagram  Latency=0  AutoFrameSizeCalculation=off
      link override Signal_Limit/_maxval: Value=KOUTP_WinLROpenedSta_pct_maxval
      link override Signal_Limit/_minval: Value=KOUTP_WinLROpenedSta_pct_minval
      link override Signal_Override/_ovrdflg: Value=KOUTP_WinLROpenedSta_pct_ovrdflg
      link override Signal_Override/_ovrdval: Value=KOUTP_WinLROpenedSta_pct_ovrdval
  VBCM_WinRFOpenedSta_pct_Inproc : FVT_lib/outp/OverrideAndLimit  SystemSampleTime=-1  VariantActivationTime=update diagram  Latency=0  AutoFrameSizeCalculation=off
      link override Signal_Limit/_maxval: Value=KOUTP_WinRFOpenedSta_pct_maxval
      link override Signal_Limit/_minval: Value=KOUTP_WinRFOpenedSta_pct_minval
      link override Signal_Override/_ovrdflg: Value=KOUTP_WinRFOpenedSta_pct_ovrdflg
      link override Signal_Override/_ovrdval: Value=KOUTP_WinRFOpenedSta_pct_ovrdval
  VBCM_WinRROpenedSta_pct_Inproc : FVT_lib/outp/OverrideAndLimit  SystemSampleTime=-1  VariantActivationTime=update diagram  Latency=0  AutoFrameSizeCalculation=off
      link override Signal_Limit/_maxval: Value=KOUTP_WinRROpenedSta_pct_maxval
      link override Signal_Limit/_minval: Value=KOUTP_WinRROpenedSta_pct_minval
      link override Signal_Override/_ovrdflg: Value=KOUTP_WinRROpenedSta_pct_ovrdflg
      link override Signal_Override/_ovrdval: Value=KOUTP_WinRROpenedSta_pct_ovrdval
  VBCM_WiperFixMode_flg_Inproc : FVT_lib/outp/OverrideAndLimit  SystemSampleTime=-1  VariantActivationTime=update diagram  Latency=0  AutoFrameSizeCalculation=off
      link override Signal_Limit/_maxval: Value=KOUTP_WiperFixMode_flg_maxval
      link override Signal_Limit/_minval: Value=KOUTP_WiperFixMode_flg_minval
      link override Signal_Override/_ovrdflg: Value=KOUTP_WiperFixMode_flg_ovrdflg
      link override Signal_Override/_ovrdval: Value=KOUTP_WiperFixMode_flg_ovrdval
  VBCM_fUnlockSingle_flg_Inproc : FVT_lib/outp/OverrideAndLimit  SystemSampleTime=-1  VariantActivationTime=update diagram  Latency=0  AutoFrameSizeCalculation=off
      link override Signal_Limit/_maxval: Value=KOUTP_fUnlockSingle_flg_maxval
      link override Signal_Limit/_minval: Value=KOUTP_fUnlockSingle_flg_minval
      link override Signal_Override/_ovrdflg: Value=KOUTP_fUnlockSingle_flg_ovrdflg
      link override Signal_Override/_ovrdval: Value=KOUTP_fUnlockSingle_flg_ovrdval
  VDDM_5vAPS1PwrErrDTC_raw32_Inproc : FVT_lib/outp/OverrideAndLimit  SystemSampleTime=-1  VariantActivationTime=update diagram  Latency=0  AutoFrameSizeCalculation=off
      link override Signal_Limit/_maxval: Value=KOUTP_5vAPS1PwrErrDTC_raw32_maxval
      link override Signal_Limit/_minval: Value=KOUTP_5vAPS1PwrErrDTC_raw32_minval
      link override Signal_Override/_ovrdflg: Value=KOUTP_5vAPS1PwrErrDTC_raw32_ovrdflg
      link override Signal_Override/_ovrdval: Value=KOUTP_5vAPS1PwrErrDTC_raw32_ovrdval
  VDDM_5vAPS2PwrErrDTC_raw32_Inproc : FVT_lib/outp/OverrideAndLimit  SystemSampleTime=-1  VariantActivationTime=update diagram  Latency=0  AutoFrameSizeCalculation=off
      link override Signal_Limit/_maxval: Value=KOUTP_5vAPS2PwrErrDTC_raw32_maxval
      link override Signal_Limit/_minval: Value=KOUTP_5vAPS2PwrErrDTC_raw32_minval
      link override Signal_Override/_ovrdflg: Value=KOUTP_5vAPS2PwrErrDTC_raw32_ovrdflg
      link override Signal_Override/_ovrdval: Value=KOUTP_5vAPS2PwrErrDTC_raw32_ovrdval
  VDDM_ACCAccelCmdErrDetDTC_raw32_Inproc : FVT_lib/outp/OverrideAndLimit  SystemSampleTime=-1  VariantActivationTime=update diagram  Latency=0  AutoFrameSizeCalculation=off
      link override Signal_Limit/_maxval: Value=KOUTP_ACCAccelCmdErrDetDTC_raw32_maxval
      link override Signal_Limit/_minval: Value=KOUTP_ACCAccelCmdErrDetDTC_raw32_minval
      link override Signal_Override/_ovrdflg: Value=KOUTP_ACCAccelCmdErrDetDTC_raw32_ovrdflg
      link override Signal_Override/_ovrdval: Value=KOUTP_ACCAccelCmdErrDetDTC_raw32_ovrdval
  VDDM_ACCMalfuncDetDTC_raw32_Inproc : FVT_lib/outp/OverrideAndLimit  SystemSampleTime=-1  VariantActivationTime=update diagram  Latency=0  AutoFrameSizeCalculation=off
      link override Signal_Limit/_maxval: Value=KOUTP_ACCMalfuncDetDTC_raw32_maxval
      link override Signal_Limit/_minval: Value=KOUTP_ACCMalfuncDetDTC_raw32_minval
      link override Signal_Override/_ovrdflg: Value=KOUTP_ACCMalfuncDetDTC_raw32_ovrdflg
      link override Signal_Override/_ovrdval: Value=KOUTP_ACCMalfuncDetDTC_raw32_ovrdval
  VDDM_APS1SigOoRDTC_raw32_Inproc : FVT_lib/outp/OverrideAndLimit  SystemSampleTime=-1  VariantActivationTime=update diagram  Latency=0  AutoFrameSizeCalculation=off
      link override Signal_Limit/_maxval: Value=KOUTP_APS1SigOoRDTC_raw32_maxval
      link override Signal_Limit/_minval: Value=KOUTP_APS1SigOoRDTC_raw32_minval
      link override Signal_Override/_ovrdflg: Value=KOUTP_APS1SigOoRDTC_raw32_ovrdflg
      link override Signal_Override/_ovrdval: Value=KOUTP_APS1SigOoRDTC_raw32_ovrdval
  VDDM_APS2SigOoRDTC_raw32_Inproc : FVT_lib/outp/OverrideAndLimit  SystemSampleTime=-1  VariantActivationTime=update diagram  Latency=0  AutoFrameSizeCalculation=off
      link override Signal_Limit/_maxval: Value=KOUTP_APS2SigOoRDTC_raw32_maxval
      link override Signal_Limit/_minval: Value=KOUTP_APS2SigOoRDTC_raw32_minval
      link override Signal_Override/_ovrdflg: Value=KOUTP_APS2SigOoRDTC_raw32_ovrdflg
      link override Signal_Override/_ovrdval: Value=KOUTP_APS2SigOoRDTC_raw32_ovrdval
  VDDM_APSCorrErrDTC_raw32_Inproc : FVT_lib/outp/OverrideAndLimit  SystemSampleTime=-1  VariantActivationTime=update diagram  Latency=0  AutoFrameSizeCalculation=off
      link override Signal_Limit/_maxval: Value=KOUTP_APSCorrErrDTC_raw32_maxval
      link override Signal_Limit/_minval: Value=KOUTP_APSCorrErrDTC_raw32_minval
      link override Signal_Override/_ovrdflg: Value=KOUTP_APSCorrErrDTC_raw32_ovrdflg
      link override Signal_Override/_ovrdval: Value=KOUTP_APSCorrErrDTC_raw32_ovrdval
  VDDM_BMSRdyDTC_raw32_Inproc : FVT_lib/outp/OverrideAndLimit  SystemSampleTime=-1  VariantActivationTime=update diagram  Latency=0  AutoFrameSizeCalculation=off
      link override Signal_Limit/_maxval: Value=KOUTP_BMSRdyDTC_raw32_maxval
      link override Signal_Limit/_minval: Value=KOUTP_BMSRdyDTC_raw32_minval
      link override Signal_Override/_ovrdflg: Value=KOUTP_BMSRdyDTC_raw32_ovrdflg
      link override Signal_Override/_ovrdval: Value=KOUTP_BMSRdyDTC_raw32_ovrdval
  VDDM_BMSSigErrDetDTC_raw32_Inproc : FVT_lib/outp/OverrideAndLimit  SystemSampleTime=-1  VariantActivationTime=update diagram  Latency=0  AutoFrameSizeCalculation=off
      link override Signal_Limit/_maxval: Value=KOUTP_BMSSigErrDetDTC_raw32_maxval
      link override Signal_Limit/_minval: Value=KOUTP_BMSSigErrDetDTC_raw32_minval
      link override Signal_Override/_ovrdflg: Value=KOUTP_BMSSigErrDetDTC_raw32_ovrdflg
      link override Signal_Override/_ovrdval: Value=KOUTP_BMSSigErrDetDTC_raw32_ovrdval
  VDDM_BrkSWErrDTC_raw32_Inproc : FVT_lib/outp/OverrideAndLimit  SystemSampleTime=-1  VariantActivationTime=update diagram  Latency=0  AutoFrameSizeCalculation=off
      link override Signal_Limit/_maxval: Value=KOUTP_BrkSWErrDTC_raw32_maxval
      link override Signal_Limit/_minval: Value=KOUTP_BrkSWErrDTC_raw32_minval
      link override Signal_Override/_ovrdflg: Value=KOUTP_BrkSWErrDTC_raw32_ovrdflg
      link override Signal_Override/_ovrdval: Value=KOUTP_BrkSWErrDTC_raw32_ovrdval
  VDDM_BrkSWNoBacDTC_raw32_Inproc : FVT_lib/outp/OverrideAndLimit  SystemSampleTime=-1  VariantActivationTime=update diagram  Latency=0  AutoFrameSizeCalculation=off
      link override Signal_Limit/_maxval: Value=KOUTP_BrkSWNoBacDTC_raw32_maxval
      link override Signal_Limit/_minval: Value=KOUTP_BrkSWNoBacDTC_raw32_minval
      link override Signal_Override/_ovrdflg: Value=KOUTP_BrkSWNoBacDTC_raw32_ovrdflg
      link override Signal_Override/_ovrdval: Value=KOUTP_BrkSWNoBacDTC_raw32_ovrdval
  VDDM_C1ABM1CSDTC_raw32_Inproc : FVT_lib/outp/OverrideAndLimit  SystemSampleTime=-1  VariantActivationTime=update diagram  Latency=0  AutoFrameSizeCalculation=off
      link override Signal_Limit/_maxval: Value=KOUTP_C1ABM1CSDTC_raw32_maxval
      link override Signal_Limit/_minval: Value=KOUTP_C1ABM1CSDTC_raw32_minval
      link override Signal_Override/_ovrdflg: Value=KOUTP_C1ABM1CSDTC_raw32_ovrdflg
      link override Signal_Override/_ovrdval: Value=KOUTP_C1ABM1CSDTC_raw32_ovrdval
  VDDM_C1ABM1LCDTC_raw32_Inproc : FVT_lib/outp/OverrideAndLimit  SystemSampleTime=-1  VariantActivationTime=update diagram  Latency=0  AutoFrameSizeCalculation=off
      link override Signal_Limit/_maxval: Value=KOUTP_C1ABM1LCDTC_raw32_maxval
      link override Signal_Limit/_minval: Value=KOUTP_C1ABM1LCDTC_raw32_minval
      link override Signal_Override/_ovrdflg: Value=KOUTP_C1ABM1LCDTC_raw32_ovrdflg
      link override Signal_Override/_ovrdval: Value=KOUTP_C1ABM1LCDTC_raw32_ovrdval
  VDDM_C1ABM1RCDTC_raw32_Inproc : FVT_lib/outp/OverrideAndLimit  SystemSampleTime=-1  VariantActivationTime=update diagram  Latency=0  AutoFrameSizeCalculation=off
      link override Signal_Limit/_maxval: Value=KOUTP_C1ABM1RCDTC_raw32_maxval
      link override Signal_Limit/_minval: Value=KOUTP_C1ABM1RCDTC_raw32_minval
      link override Signal_Override/_ovrdflg: Value=KOUTP_C1ABM1RCDTC_raw32_ovrdflg
      link override Signal_Override/_ovrdval: Value=KOUTP_C1ABM1RCDTC_raw32_ovrdval
  VDDM_C1EPAS2LCDTC_raw32_Inproc : FVT_lib/outp/OverrideAndLimit  SystemSampleTime=-1  VariantActivationTime=update diagram  Latency=0  AutoFrameSizeCalculation=off
      link override Signal_Limit/_maxval: Value=KOUTP_C1EPAS2LCDTC_raw32_maxval
      link override Signal_Limit/_minval: Value=KOUTP_C1EPAS2LCDTC_raw32_minval
      link override Signal_Override/_ovrdflg: Value=KOUTP_C1EPAS2LCDTC_raw32_ovrdflg
      link override Signal_Override/_ovrdval: Value=KOUTP_C1EPAS2LCDTC_raw32_ovrdval
  VDDM_C3BMS1CSDTC_raw32_Inproc : FVT_lib/outp/OverrideAndLimit  SystemSampleTime=-1  VariantActivationTime=update diagram  Latency=0  AutoFrameSizeCalculation=off
      link override Signal_Limit/_maxval: Value=KOUTP_C3BMS1CSDTC_raw32_maxval
      link override Signal_Limit/_minval: Value=KOUTP_C3BMS1CSDTC_raw32_minval
      link override Signal_Override/_ovrdflg: Value=KOUTP_C3BMS1CSDTC_raw32_ovrdflg
      link override Signal_Override/_ovrdval: Value=KOUTP_C3BMS1CSDTC_raw32_ovrdval
  VDDM_C3BMS1LCDTC_raw32_Inproc : FVT_lib/outp/OverrideAndLimit  SystemSampleTime=-1  VariantActivationTime=update diagram  Latency=0  AutoFrameSizeCalculation=off
      link override Signal_Limit/_maxval: Value=KOUTP_C3BMS1LCDTC_raw32_maxval
      link override Signal_Limit/_minval: Value=KOUTP_C3BMS1LCDTC_raw32_minval
      link override Signal_Override/_ovrdflg: Value=KOUTP_C3BMS1LCDTC_raw32_ovrdflg
      link override Signal_Override/_ovrdval: Value=KOUTP_C3BMS1LCDTC_raw32_ovrdval
  VDDM_C3BMS1RCDTC_raw32_Inproc : FVT_lib/outp/OverrideAndLimit  SystemSampleTime=-1  VariantActivationTime=update diagram  Latency=0  AutoFrameSizeCalculation=off
      link override Signal_Limit/_maxval: Value=KOUTP_C3BMS1RCDTC_raw32_maxval
      link override Signal_Limit/_minval: Value=KOUTP_C3BMS1RCDTC_raw32_minval
      link override Signal_Override/_ovrdflg: Value=KOUTP_C3BMS1RCDTC_raw32_ovrdflg
      link override Signal_Override/_ovrdval: Value=KOUTP_C3BMS1RCDTC_raw32_ovrdval
  VDDM_C3BMS6CSDTC_raw32_Inproc : FVT_lib/outp/OverrideAndLimit  SystemSampleTime=-1  VariantActivationTime=update diagram  Latency=0  AutoFrameSizeCalculation=off
      link override Signal_Limit/_maxval: Value=KOUTP_C3BMS6CSDTC_raw32_maxval
      link override Signal_Limit/_minval: Value=KOUTP_C3BMS6CSDTC_raw32_minval
      link override Signal_Override/_ovrdflg: Value=KOUTP_C3BMS6CSDTC_raw32_ovrdflg
      link override Signal_Override/_ovrdval: Value=KOUTP_C3BMS6CSDTC_raw32_ovrdval
  VDDM_C3BMS6LCDTC_raw32_Inproc : FVT_lib/outp/OverrideAndLimit  SystemSampleTime=-1  VariantActivationTime=update diagram  Latency=0  AutoFrameSizeCalculation=off
      link override Signal_Limit/_maxval: Value=KOUTP_C3BMS6LCDTC_raw32_maxval
      link override Signal_Limit/_minval: Value=KOUTP_C3BMS6LCDTC_raw32_minval
      link override Signal_Override/_ovrdflg: Value=KOUTP_C3BMS6LCDTC_raw32_ovrdflg
      link override Signal_Override/_ovrdval: Value=KOUTP_C3BMS6LCDTC_raw32_ovrdval
  VDDM_C3BMS6RCDTC_raw32_Inproc : FVT_lib/outp/OverrideAndLimit  SystemSampleTime=-1  VariantActivationTime=update diagram  Latency=0  AutoFrameSizeCalculation=off
      link override Signal_Limit/_maxval: Value=KOUTP_C3BMS6RCDTC_raw32_maxval
      link override Signal_Limit/_minval: Value=KOUTP_C3BMS6RCDTC_raw32_minval
      link override Signal_Override/_ovrdflg: Value=KOUTP_C3BMS6RCDTC_raw32_ovrdflg
      link override Signal_Override/_ovrdval: Value=KOUTP_C3BMS6RCDTC_raw32_ovrdval
  VDDM_C3CCU1CSDTC_raw32_Inproc : FVT_lib/outp/OverrideAndLimit  SystemSampleTime=-1  VariantActivationTime=update diagram  Latency=0  AutoFrameSizeCalculation=off
      link override Signal_Limit/_maxval: Value=KOUTP_C3CCU1CSDTC_raw32_maxval
      link override Signal_Limit/_minval: Value=KOUTP_C3CCU1CSDTC_raw32_minval
      link override Signal_Override/_ovrdflg: Value=KOUTP_C3CCU1CSDTC_raw32_ovrdflg
      link override Signal_Override/_ovrdval: Value=KOUTP_C3CCU1CSDTC_raw32_ovrdval
  VDDM_C3CCU1LCDTC_raw32_Inproc : FVT_lib/outp/OverrideAndLimit  SystemSampleTime=-1  VariantActivationTime=update diagram  Latency=0  AutoFrameSizeCalculation=off
      link override Signal_Limit/_maxval: Value=KOUTP_C3CCU1LCDTC_raw32_maxval
      link override Signal_Limit/_minval: Value=KOUTP_C3CCU1LCDTC_raw32_minval
      link override Signal_Override/_ovrdflg: Value=KOUTP_C3CCU1LCDTC_raw32_ovrdflg
      link override Signal_Override/_ovrdval: Value=KOUTP_C3CCU1LCDTC_raw32_ovrdval
  VDDM_C3CCU1RCDTC_raw32_Inproc : FVT_lib/outp/OverrideAndLimit  SystemSampleTime=-1  VariantActivationTime=update diagram  Latency=0  AutoFrameSizeCalculation=off
      link override Signal_Limit/_maxval: Value=KOUTP_C3CCU1RCDTC_raw32_maxval
      link override Signal_Limit/_minval: Value=KOUTP_C3CCU1RCDTC_raw32_minval
      link override Signal_Override/_ovrdflg: Value=KOUTP_C3CCU1RCDTC_raw32_ovrdflg
      link override Signal_Override/_ovrdval: Value=KOUTP_C3CCU1RCDTC_raw32_ovrdval
  VDDM_C3CCU2CSDTC_raw32_Inproc : FVT_lib/outp/OverrideAndLimit  SystemSampleTime=-1  VariantActivationTime=update diagram  Latency=0  AutoFrameSizeCalculation=off
      link override Signal_Limit/_maxval: Value=KOUTP_C3CCU2CSDTC_raw32_maxval
      link override Signal_Limit/_minval: Value=KOUTP_C3CCU2CSDTC_raw32_minval
      link override Signal_Override/_ovrdflg: Value=KOUTP_C3CCU2CSDTC_raw32_ovrdflg
      link override Signal_Override/_ovrdval: Value=KOUTP_C3CCU2CSDTC_raw32_ovrdval
  VDDM_C3CCU2LCDTC_raw32_Inproc : FVT_lib/outp/OverrideAndLimit  SystemSampleTime=-1  VariantActivationTime=update diagram  Latency=0  AutoFrameSizeCalculation=off
      link override Signal_Limit/_maxval: Value=KOUTP_C3CCU2LCDTC_raw32_maxval
      link override Signal_Limit/_minval: Value=KOUTP_C3CCU2LCDTC_raw32_minval
      link override Signal_Override/_ovrdflg: Value=KOUTP_C3CCU2LCDTC_raw32_ovrdflg
      link override Signal_Override/_ovrdval: Value=KOUTP_C3CCU2LCDTC_raw32_ovrdval
  VDDM_C3CCU2RCDTC_raw32_Inproc : FVT_lib/outp/OverrideAndLimit  SystemSampleTime=-1  VariantActivationTime=update diagram  Latency=0  AutoFrameSizeCalculation=off
      link override Signal_Limit/_maxval: Value=KOUTP_C3CCU2RCDTC_raw32_maxval
      link override Signal_Limit/_minval: Value=KOUTP_C3CCU2RCDTC_raw32_minval
      link override Signal_Override/_ovrdflg: Value=KOUTP_C3CCU2RCDTC_raw32_ovrdflg
      link override Signal_Override/_ovrdval: Value=KOUTP_C3CCU2RCDTC_raw32_ovrdval
  VDDM_CAN1BusErrorDTC_raw32_Inproc : FVT_lib/outp/OverrideAndLimit  SystemSampleTime=-1  VariantActivationTime=update diagram  Latency=0  AutoFrameSizeCalculation=off
      link override Signal_Limit/_maxval: Value=KOUTP_CAN1BusErrorDTC_raw32_maxval
      link override Signal_Limit/_minval: Value=KOUTP_CAN1BusErrorDTC_raw32_minval
      link override Signal_Override/_ovrdflg: Value=KOUTP_CAN1BusErrorDTC_raw32_ovrdflg
      link override Signal_Override/_ovrdval: Value=KOUTP_CAN1BusErrorDTC_raw32_ovrdval
  VDDM_CAN1BusOffDTC_raw32_Inproc : FVT_lib/outp/OverrideAndLimit  SystemSampleTime=-1  VariantActivationTime=update diagram  Latency=0  AutoFrameSizeCalculation=off
      link override Signal_Limit/_maxval: Value=KOUTP_CAN1BusOffDTC_raw32_maxval
      link override Signal_Limit/_minval: Value=KOUTP_CAN1BusOffDTC_raw32_minval
      link override Signal_Override/_ovrdflg: Value=KOUTP_CAN1BusOffDTC_raw32_ovrdflg
      link override Signal_Override/_ovrdval: Value=KOUTP_CAN1BusOffDTC_raw32_ovrdval
  VDDM_CAN2BusErrorDTC_raw32_Inproc : FVT_lib/outp/OverrideAndLimit  SystemSampleTime=-1  VariantActivationTime=update diagram  Latency=0  AutoFrameSizeCalculation=off
      link override Signal_Limit/_maxval: Value=KOUTP_CAN2BusErrorDTC_raw32_maxval
      link override Signal_Limit/_minval: Value=KOUTP_CAN2BusErrorDTC_raw32_minval
      link override Signal_Override/_ovrdflg: Value=KOUTP_CAN2BusErrorDTC_raw32_ovrdflg
      link override Signal_Override/_ovrdval: Value=KOUTP_CAN2BusErrorDTC_raw32_ovrdval
  VDDM_CAN2BusOffDTC_raw32_Inproc : FVT_lib/outp/OverrideAndLimit  SystemSampleTime=-1  VariantActivationTime=update diagram  Latency=0  AutoFrameSizeCalculation=off
      link override Signal_Limit/_maxval: Value=KOUTP_CAN2BusOffDTC_raw32_maxval
      link override Signal_Limit/_minval: Value=KOUTP_CAN2BusOffDTC_raw32_minval
      link override Signal_Override/_ovrdflg: Value=KOUTP_CAN2BusOffDTC_raw32_ovrdflg
      link override Signal_Override/_ovrdval: Value=KOUTP_CAN2BusOffDTC_raw32_ovrdval
  VDDM_CAN3BusErrorDTC_raw32_Inproc : FVT_lib/outp/OverrideAndLimit  SystemSampleTime=-1  VariantActivationTime=update diagram  Latency=0  AutoFrameSizeCalculation=off
      link override Signal_Limit/_maxval: Value=KOUTP_CAN3BusErrorDTC_raw32_maxval
      link override Signal_Limit/_minval: Value=KOUTP_CAN3BusErrorDTC_raw32_minval
      link override Signal_Override/_ovrdflg: Value=KOUTP_CAN3BusErrorDTC_raw32_ovrdflg
      link override Signal_Override/_ovrdval: Value=KOUTP_CAN3BusErrorDTC_raw32_ovrdval
  VDDM_CAN3BusOffDTC_raw32_Inproc : FVT_lib/outp/OverrideAndLimit  SystemSampleTime=-1  VariantActivationTime=update diagram  Latency=0  AutoFrameSizeCalculation=off
      link override Signal_Limit/_maxval: Value=KOUTP_CAN3BusOffDTC_raw32_maxval
      link override Signal_Limit/_minval: Value=KOUTP_CAN3BusOffDTC_raw32_minval
      link override Signal_Override/_ovrdflg: Value=KOUTP_CAN3BusOffDTC_raw32_ovrdflg
      link override Signal_Override/_ovrdval: Value=KOUTP_CAN3BusOffDTC_raw32_ovrdval
  VDDM_CAN4BusErrorDTC_raw32_Inproc : FVT_lib/outp/OverrideAndLimit  SystemSampleTime=-1  VariantActivationTime=update diagram  Latency=0  AutoFrameSizeCalculation=off
      link override Signal_Limit/_maxval: Value=KOUTP_CAN4BusErrorDTC_raw32_maxval
      link override Signal_Limit/_minval: Value=KOUTP_CAN4BusErrorDTC_raw32_minval
      link override Signal_Override/_ovrdflg: Value=KOUTP_CAN4BusErrorDTC_raw32_ovrdflg
      link override Signal_Override/_ovrdval: Value=KOUTP_CAN4BusErrorDTC_raw32_ovrdval
  VDDM_CAN4BusOffDTC_raw32_Inproc : FVT_lib/outp/OverrideAndLimit  SystemSampleTime=-1  VariantActivationTime=update diagram  Latency=0  AutoFrameSizeCalculation=off
      link override Signal_Limit/_maxval: Value=KOUTP_CAN4BusOffDTC_raw32_maxval
      link override Signal_Limit/_minval: Value=KOUTP_CAN4BusOffDTC_raw32_minval
      link override Signal_Override/_ovrdflg: Value=KOUTP_CAN4BusOffDTC_raw32_ovrdflg
      link override Signal_Override/_ovrdval: Value=KOUTP_CAN4BusOffDTC_raw32_ovrdval
  VDDM_CAN5BusErrorDTC_raw32_Inproc : FVT_lib/outp/OverrideAndLimit  SystemSampleTime=-1  VariantActivationTime=update diagram  Latency=0  AutoFrameSizeCalculation=off
      link override Signal_Limit/_maxval: Value=KOUTP_CAN5BusErrorDTC_raw32_maxval
      link override Signal_Limit/_minval: Value=KOUTP_CAN5BusErrorDTC_raw32_minval
      link override Signal_Override/_ovrdflg: Value=KOUTP_CAN5BusErrorDTC_raw32_ovrdflg
      link override Signal_Override/_ovrdval: Value=KOUTP_CAN5BusErrorDTC_raw32_ovrdval
  VDDM_CAN5BusOffDTC_raw32_Inproc : FVT_lib/outp/OverrideAndLimit  SystemSampleTime=-1  VariantActivationTime=update diagram  Latency=0  AutoFrameSizeCalculation=off
      link override Signal_Limit/_maxval: Value=KOUTP_CAN5BusOffDTC_raw32_maxval
      link override Signal_Limit/_minval: Value=KOUTP_CAN5BusOffDTC_raw32_minval
      link override Signal_Override/_ovrdflg: Value=KOUTP_CAN5BusOffDTC_raw32_ovrdflg
      link override Signal_Override/_ovrdval: Value=KOUTP_CAN5BusOffDTC_raw32_ovrdval
  VDDM_CAN6BusErrorDTC_raw32_Inproc : FVT_lib/outp/OverrideAndLimit  SystemSampleTime=-1  VariantActivationTime=update diagram  Latency=0  AutoFrameSizeCalculation=off
      link override Signal_Limit/_maxval: Value=KOUTP_CAN6BusErrorDTC_raw32_maxval
      link override Signal_Limit/_minval: Value=KOUTP_CAN6BusErrorDTC_raw32_minval
      link override Signal_Override/_ovrdflg: Value=KOUTP_CAN6BusErrorDTC_raw32_ovrdflg
      link override Signal_Override/_ovrdval: Value=KOUTP_CAN6BusErrorDTC_raw32_ovrdval
  VDDM_CAN6BusOffDTC_raw32_Inproc : FVT_lib/outp/OverrideAndLimit  SystemSampleTime=-1  VariantActivationTime=update diagram  Latency=0  AutoFrameSizeCalculation=off
      link override Signal_Limit/_maxval: Value=KOUTP_CAN6BusOffDTC_raw32_maxval
      link override Signal_Limit/_minval: Value=KOUTP_CAN6BusOffDTC_raw32_minval
      link override Signal_Override/_ovrdflg: Value=KOUTP_CAN6BusOffDTC_raw32_ovrdflg
      link override Signal_Override/_ovrdval: Value=KOUTP_CAN6BusOffDTC_raw32_ovrdval
  VDDM_CCMalfuncDetDTC_raw32_Inproc : FVT_lib/outp/OverrideAndLimit  SystemSampleTime=-1  VariantActivationTime=update diagram  Latency=0  AutoFrameSizeCalculation=off
      link override Signal_Limit/_maxval: Value=KOUTP_CCMalfuncDetDTC_raw32_maxval
      link override Signal_Limit/_minval: Value=KOUTP_CCMalfuncDetDTC_raw32_minval
      link override Signal_Override/_ovrdflg: Value=KOUTP_CCMalfuncDetDTC_raw32_ovrdflg
      link override Signal_Override/_ovrdval: Value=KOUTP_CCMalfuncDetDTC_raw32_ovrdval
  VDDM_CCUSigErrDetDTC_raw32_Inproc : FVT_lib/outp/OverrideAndLimit  SystemSampleTime=-1  VariantActivationTime=update diagram  Latency=0  AutoFrameSizeCalculation=off
      link override Signal_Limit/_maxval: Value=KOUTP_CCUSigErrDetDTC_raw32_maxval
      link override Signal_Limit/_minval: Value=KOUTP_CCUSigErrDetDTC_raw32_minval
      link override Signal_Override/_ovrdflg: Value=KOUTP_CCUSigErrDetDTC_raw32_ovrdflg
      link override Signal_Override/_ovrdval: Value=KOUTP_CCUSigErrDetDTC_raw32_ovrdval
  VDDM_DCDC4PreDTC_raw32_Inproc : FVT_lib/outp/OverrideAndLimit  SystemSampleTime=-1  VariantActivationTime=update diagram  Latency=0  AutoFrameSizeCalculation=off
      link override Signal_Limit/_maxval: Value=KOUTP_DCDC4PreDTC_raw32_maxval
      link override Signal_Limit/_minval: Value=KOUTP_DCDC4PreDTC_raw32_minval
      link override Signal_Override/_ovrdflg: Value=KOUTP_DCDC4PreDTC_raw32_ovrdflg
      link override Signal_Override/_ovrdval: Value=KOUTP_DCDC4PreDTC_raw32_ovrdval
  VDDM_DCDCDisDTC_raw32_Inproc : FVT_lib/outp/OverrideAndLimit  SystemSampleTime=-1  VariantActivationTime=update diagram  Latency=0  AutoFrameSizeCalculation=off
      link override Signal_Limit/_maxval: Value=KOUTP_DCDCDisDTC_raw32_maxval
      link override Signal_Limit/_minval: Value=KOUTP_DCDCDisDTC_raw32_minval
      link override Signal_Override/_ovrdflg: Value=KOUTP_DCDCDisDTC_raw32_ovrdflg
      link override Signal_Override/_ovrdval: Value=KOUTP_DCDCDisDTC_raw32_ovrdval
  VDDM_DCDCEnaDTC_raw32_Inproc : FVT_lib/outp/OverrideAndLimit  SystemSampleTime=-1  VariantActivationTime=update diagram  Latency=0  AutoFrameSizeCalculation=off
      link override Signal_Limit/_maxval: Value=KOUTP_DCDCEnaDTC_raw32_maxval
      link override Signal_Limit/_minval: Value=KOUTP_DCDCEnaDTC_raw32_minval
      link override Signal_Override/_ovrdflg: Value=KOUTP_DCDCEnaDTC_raw32_ovrdflg
      link override Signal_Override/_ovrdval: Value=KOUTP_DCDCEnaDTC_raw32_ovrdval
  VDDM_DTCDetect_enum_Inproc : FVT_lib/outp/OverrideAndLimit  SystemSampleTime=-1  VariantActivationTime=update diagram  Latency=0  AutoFrameSizeCalculation=off
      link override Signal_Limit/_maxval: Value=KOUTP_DTCDetect_enum_maxval
      link override Signal_Limit/_minval: Value=KOUTP_DTCDetect_enum_minval
      link override Signal_Override/_ovrdflg: Value=KOUTP_DTCDetect_enum_ovrdflg
      link override Signal_Override/_ovrdval: Value=KOUTP_DTCDetect_enum_ovrdval
  VDDM_DiagFLTSDTC_raw32_Inproc : FVT_lib/outp/OverrideAndLimit  SystemSampleTime=-1  VariantActivationTime=update diagram  Latency=0  AutoFrameSizeCalculation=off
      link override Signal_Limit/_maxval: Value=KOUTP_DiagFLTSDTC_raw32_maxval
      link override Signal_Limit/_minval: Value=KOUTP_DiagFLTSDTC_raw32_minval
      link override Signal_Override/_ovrdflg: Value=KOUTP_DiagFLTSDTC_raw32_ovrdflg
      link override Signal_Override/_ovrdval: Value=KOUTP_DiagFLTSDTC_raw32_ovrdval
  VDDM_DiagFRTSDTC_raw32_Inproc : FVT_lib/outp/OverrideAndLimit  SystemSampleTime=-1  VariantActivationTime=update diagram  Latency=0  AutoFrameSizeCalculation=off
      link override Signal_Limit/_maxval: Value=KOUTP_DiagFRTSDTC_raw32_maxval
      link override Signal_Limit/_minval: Value=KOUTP_DiagFRTSDTC_raw32_minval
      link override Signal_Override/_ovrdflg: Value=KOUTP_DiagFRTSDTC_raw32_ovrdflg
      link override Signal_Override/_ovrdval: Value=KOUTP_DiagFRTSDTC_raw32_ovrdval
  VDDM_DiagHCrashDTC_raw32_Inproc : FVT_lib/outp/OverrideAndLimit  SystemSampleTime=-1  VariantActivationTime=update diagram  Latency=0  AutoFrameSizeCalculation=off
      link override Signal_Limit/_maxval: Value=KOUTP_DiagHCrashDTC_raw32_maxval
      link override Signal_Limit/_minval: Value=KOUTP_DiagHCrashDTC_raw32_minval
      link override Signal_Override/_ovrdflg: Value=KOUTP_DiagHCrashDTC_raw32_ovrdflg
      link override Signal_Override/_ovrdval: Value=KOUTP_DiagHCrashDTC_raw32_ovrdval
  VDDM_DiagRLTSDTC_raw32_Inproc : FVT_lib/outp/OverrideAndLimit  SystemSampleTime=-1  VariantActivationTime=update diagram  Latency=0  AutoFrameSizeCalculation=off
      link override Signal_Limit/_maxval: Value=KOUTP_DiagRLTSDTC_raw32_maxval
      link override Signal_Limit/_minval: Value=KOUTP_DiagRLTSDTC_raw32_minval
      link override Signal_Override/_ovrdflg: Value=KOUTP_DiagRLTSDTC_raw32_ovrdflg
      link override Signal_Override/_ovrdval: Value=KOUTP_DiagRLTSDTC_raw32_ovrdval
  VDDM_DiagRRTSDTC_raw32_Inproc : FVT_lib/outp/OverrideAndLimit  SystemSampleTime=-1  VariantActivationTime=update diagram  Latency=0  AutoFrameSizeCalculation=off
      link override Signal_Limit/_maxval: Value=KOUTP_DiagRRTSDTC_raw32_maxval
      link override Signal_Limit/_minval: Value=KOUTP_DiagRRTSDTC_raw32_minval
      link override Signal_Override/_ovrdflg: Value=KOUTP_DiagRRTSDTC_raw32_ovrdflg
      link override Signal_Override/_ovrdval: Value=KOUTP_DiagRRTSDTC_raw32_ovrdval
  VDDM_DisengagePFail_flg_Inproc : FVT_lib/outp/OverrideAndLimit  SystemSampleTime=-1  VariantActivationTime=update diagram  Latency=0  AutoFrameSizeCalculation=off
      link override Signal_Limit/_maxval: Value=KOUTP_DisengagePFail_flg_maxval
      link override Signal_Limit/_minval: Value=KOUTP_DisengagePFail_flg_minval
      link override Signal_Override/_ovrdflg: Value=KOUTP_DisengagePFail_flg_ovrdflg
      link override Signal_Override/_ovrdval: Value=KOUTP_DisengagePFail_flg_ovrdval
  VDDM_DrStSWDTC_raw32_Inproc : FVT_lib/outp/OverrideAndLimit  SystemSampleTime=-1  VariantActivationTime=update diagram  Latency=0  AutoFrameSizeCalculation=off
      link override Signal_Limit/_maxval: Value=KOUTP_DrStSWDTC_raw32_maxval
      link override Signal_Limit/_minval: Value=KOUTP_DrStSWDTC_raw32_minval
      link override Signal_Override/_ovrdflg: Value=KOUTP_DrStSWDTC_raw32_ovrdflg
      link override Signal_Override/_ovrdval: Value=KOUTP_DrStSWDTC_raw32_ovrdval
  VDDM_EDriveSysErrShifterErr_flg_Inproc : FVT_lib/outp/OverrideAndLimit  SystemSampleTime=-1  VariantActivationTime=update diagram  Latency=0  AutoFrameSizeCalculation=off
      link override Signal_Limit/_maxval: Value=KOUTP_EDriveSysErrShifterErr_flg_maxval
      link override Signal_Limit/_minval: Value=KOUTP_EDriveSysErrShifterErr_flg_minval
      link override Signal_Override/_ovrdflg: Value=KOUTP_EDriveSysErrShifterErr_flg_ovrdflg
      link override Signal_Override/_ovrdval: Value=KOUTP_EDriveSysErrShifterErr_flg_ovrdval
  VDDM_EDriveSysErrVCUErr_flg_Inproc : FVT_lib/outp/OverrideAndLimit  SystemSampleTime=-1  VariantActivationTime=update diagram  Latency=0  AutoFrameSizeCalculation=off
      link override Signal_Limit/_maxval: Value=KOUTP_EDriveSysErrVCUErr_flg_maxval
      link override Signal_Limit/_minval: Value=KOUTP_EDriveSysErrVCUErr_flg_minval
      link override Signal_Override/_ovrdflg: Value=KOUTP_EDriveSysErrVCUErr_flg_ovrdflg
      link override Signal_Override/_ovrdval: Value=KOUTP_EDriveSysErrVCUErr_flg_ovrdval
  VDDM_EPBLockTODTC_raw32_Inproc : FVT_lib/outp/OverrideAndLimit  SystemSampleTime=-1  VariantActivationTime=update diagram  Latency=0  AutoFrameSizeCalculation=off
      link override Signal_Limit/_maxval: Value=KOUTP_EPBLockTODTC_raw32_maxval
      link override Signal_Limit/_minval: Value=KOUTP_EPBLockTODTC_raw32_minval
      link override Signal_Override/_ovrdflg: Value=KOUTP_EPBLockTODTC_raw32_ovrdflg
      link override Signal_Override/_ovrdval: Value=KOUTP_EPBLockTODTC_raw32_ovrdval
  VDDM_EPBUnlockTODTC_raw32_Inproc : FVT_lib/outp/OverrideAndLimit  SystemSampleTime=-1  VariantActivationTime=update diagram  Latency=0  AutoFrameSizeCalculation=off
      link override Signal_Limit/_maxval: Value=KOUTP_EPBUnlockTODTC_raw32_maxval
      link override Signal_Limit/_minval: Value=KOUTP_EPBUnlockTODTC_raw32_minval
      link override Signal_Override/_ovrdflg: Value=KOUTP_EPBUnlockTODTC_raw32_ovrdflg
      link override Signal_Override/_ovrdval: Value=KOUTP_EPBUnlockTODTC_raw32_ovrdval
  VDDM_ESC1CSErrDTC_raw32_Inproc : FVT_lib/outp/OverrideAndLimit  SystemSampleTime=-1  VariantActivationTime=update diagram  Latency=0  AutoFrameSizeCalculation=off
      link override Signal_Limit/_maxval: Value=KOUTP_ESC1CSErrDTC_raw32_maxval
      link override Signal_Limit/_minval: Value=KOUTP_ESC1CSErrDTC_raw32_minval
      link override Signal_Override/_ovrdflg: Value=KOUTP_ESC1CSErrDTC_raw32_ovrdflg
      link override Signal_Override/_ovrdval: Value=KOUTP_ESC1CSErrDTC_raw32_ovrdval
  VDDM_ESC1NoComDTC_raw32_Inproc : FVT_lib/outp/OverrideAndLimit  SystemSampleTime=-1  VariantActivationTime=update diagram  Latency=0  AutoFrameSizeCalculation=off
      link override Signal_Limit/_maxval: Value=KOUTP_ESC1NoComDTC_raw32_maxval
      link override Signal_Limit/_minval: Value=KOUTP_ESC1NoComDTC_raw32_minval
      link override Signal_Override/_ovrdflg: Value=KOUTP_ESC1NoComDTC_raw32_ovrdflg
      link override Signal_Override/_ovrdval: Value=KOUTP_ESC1NoComDTC_raw32_ovrdval
  VDDM_ESC1RCErrDTC_raw32_Inproc : FVT_lib/outp/OverrideAndLimit  SystemSampleTime=-1  VariantActivationTime=update diagram  Latency=0  AutoFrameSizeCalculation=off
      link override Signal_Limit/_maxval: Value=KOUTP_ESC1RCErrDTC_raw32_maxval
      link override Signal_Limit/_minval: Value=KOUTP_ESC1RCErrDTC_raw32_minval
      link override Signal_Override/_ovrdflg: Value=KOUTP_ESC1RCErrDTC_raw32_ovrdflg
      link override Signal_Override/_ovrdval: Value=KOUTP_ESC1RCErrDTC_raw32_ovrdval
  VDDM_ESC5CSErrDTC_raw32_Inproc : FVT_lib/outp/OverrideAndLimit  SystemSampleTime=-1  VariantActivationTime=update diagram  Latency=0  AutoFrameSizeCalculation=off
      link override Signal_Limit/_maxval: Value=KOUTP_ESC5CSErrDTC_raw32_maxval
      link override Signal_Limit/_minval: Value=KOUTP_ESC5CSErrDTC_raw32_minval
      link override Signal_Override/_ovrdflg: Value=KOUTP_ESC5CSErrDTC_raw32_ovrdflg
      link override Signal_Override/_ovrdval: Value=KOUTP_ESC5CSErrDTC_raw32_ovrdval
  VDDM_ESC5NoComDTC_raw32_Inproc : FVT_lib/outp/OverrideAndLimit  SystemSampleTime=-1  VariantActivationTime=update diagram  Latency=0  AutoFrameSizeCalculation=off
      link override Signal_Limit/_maxval: Value=KOUTP_ESC5NoComDTC_raw32_maxval
      link override Signal_Limit/_minval: Value=KOUTP_ESC5NoComDTC_raw32_minval
      link override Signal_Override/_ovrdflg: Value=KOUTP_ESC5NoComDTC_raw32_ovrdflg
      link override Signal_Override/_ovrdval: Value=KOUTP_ESC5NoComDTC_raw32_ovrdval
  VDDM_ESC5RCErrDTC_raw32_Inproc : FVT_lib/outp/OverrideAndLimit  SystemSampleTime=-1  VariantActivationTime=update diagram  Latency=0  AutoFrameSizeCalculation=off
      link override Signal_Limit/_maxval: Value=KOUTP_ESC5RCErrDTC_raw32_maxval
      link override Signal_Limit/_minval: Value=KOUTP_ESC5RCErrDTC_raw32_minval
      link override Signal_Override/_ovrdflg: Value=KOUTP_ESC5RCErrDTC_raw32_ovrdflg
      link override Signal_Override/_ovrdval: Value=KOUTP_ESC5RCErrDTC_raw32_ovrdval
  VDDM_ESC7CSErrDTC_raw32_Inproc : FVT_lib/outp/OverrideAndLimit  SystemSampleTime=-1  VariantActivationTime=update diagram  Latency=0  AutoFrameSizeCalculation=off
      link override Signal_Limit/_maxval: Value=KOUTP_ESC7CSErrDTC_raw32_maxval
      link override Signal_Limit/_minval: Value=KOUTP_ESC7CSErrDTC_raw32_minval
      link override Signal_Override/_ovrdflg: Value=KOUTP_ESC7CSErrDTC_raw32_ovrdflg
      link override Signal_Override/_ovrdval: Value=KOUTP_ESC7CSErrDTC_raw32_ovrdval
  VDDM_ESC7NoComDTC_raw32_Inproc : FVT_lib/outp/OverrideAndLimit  SystemSampleTime=-1  VariantActivationTime=update diagram  Latency=0  AutoFrameSizeCalculation=off
      link override Signal_Limit/_maxval: Value=KOUTP_ESC7NoComDTC_raw32_maxval
      link override Signal_Limit/_minval: Value=KOUTP_ESC7NoComDTC_raw32_minval
      link override Signal_Override/_ovrdflg: Value=KOUTP_ESC7NoComDTC_raw32_ovrdflg
      link override Signal_Override/_ovrdval: Value=KOUTP_ESC7NoComDTC_raw32_ovrdval
  VDDM_ESC7RCErrDTC_raw32_Inproc : FVT_lib/outp/OverrideAndLimit  SystemSampleTime=-1  VariantActivationTime=update diagram  Latency=0  AutoFrameSizeCalculation=off
      link override Signal_Limit/_maxval: Value=KOUTP_ESC7RCErrDTC_raw32_maxval
      link override Signal_Limit/_minval: Value=KOUTP_ESC7RCErrDTC_raw32_minval
      link override Signal_Override/_ovrdflg: Value=KOUTP_ESC7RCErrDTC_raw32_ovrdflg
      link override Signal_Override/_ovrdval: Value=KOUTP_ESC7RCErrDTC_raw32_ovrdval
  VDDM_EngagePFail_flg_Inproc : FVT_lib/outp/OverrideAndLimit  SystemSampleTime=-1  VariantActivationTime=update diagram  Latency=0  AutoFrameSizeCalculation=off
      link override Signal_Limit/_maxval: Value=KOUTP_EngagePFail_flg_maxval
      link override Signal_Limit/_minval: Value=KOUTP_EngagePFail_flg_minval
      link override Signal_Override/_ovrdflg: Value=KOUTP_EngagePFail_flg_ovrdflg
      link override Signal_Override/_ovrdval: Value=KOUTP_EngagePFail_flg_ovrdval
  VDDM_EnterNewOperCyc_flg_Inproc : FVT_lib/outp/OverrideAndLimit  SystemSampleTime=-1  VariantActivationTime=update diagram  Latency=0  AutoFrameSizeCalculation=off
      link override Signal_Limit/_maxval: Value=KOUTP_EnterNewOperCyc_flg_maxval
      link override Signal_Limit/_minval: Value=KOUTP_EnterNewOperCyc_flg_minval
      link override Signal_Override/_ovrdflg: Value=KOUTP_EnterNewOperCyc_flg_ovrdflg
      link override Signal_Override/_ovrdval: Value=KOUTP_EnterNewOperCyc_flg_ovrdval
  VDDM_FCLUSSDTC_raw32_Inproc : FVT_lib/outp/OverrideAndLimit  SystemSampleTime=-1  VariantActivationTime=update diagram  Latency=0  AutoFrameSizeCalculation=off
      link override Signal_Limit/_maxval: Value=KOUTP_FCLUSSDTC_raw32_maxval
      link override Signal_Limit/_minval: Value=KOUTP_FCLUSSDTC_raw32_minval
      link override Signal_Override/_ovrdflg: Value=KOUTP_FCLUSSDTC_raw32_ovrdflg
      link override Signal_Override/_ovrdval: Value=KOUTP_FCLUSSDTC_raw32_ovrdval
  VDDM_FCM2CSErrDTC_raw32_Inproc : FVT_lib/outp/OverrideAndLimit  SystemSampleTime=-1  VariantActivationTime=update diagram  Latency=0  AutoFrameSizeCalculation=off
      link override Signal_Limit/_maxval: Value=KOUTP_FCM2CSErrDTC_raw32_maxval
      link override Signal_Limit/_minval: Value=KOUTP_FCM2CSErrDTC_raw32_minval
      link override Signal_Override/_ovrdflg: Value=KOUTP_FCM2CSErrDTC_raw32_ovrdflg
      link override Signal_Override/_ovrdval: Value=KOUTP_FCM2CSErrDTC_raw32_ovrdval
  VDDM_FCM2NoComDTC_raw32_Inproc : FVT_lib/outp/OverrideAndLimit  SystemSampleTime=-1  VariantActivationTime=update diagram  Latency=0  AutoFrameSizeCalculation=off
      link override Signal_Limit/_maxval: Value=KOUTP_FCM2NoComDTC_raw32_maxval
      link override Signal_Limit/_minval: Value=KOUTP_FCM2NoComDTC_raw32_minval
      link override Signal_Override/_ovrdflg: Value=KOUTP_FCM2NoComDTC_raw32_ovrdflg
      link override Signal_Override/_ovrdval: Value=KOUTP_FCM2NoComDTC_raw32_ovrdval
  VDDM_FCM2RCErrDTC_raw32_Inproc : FVT_lib/outp/OverrideAndLimit  SystemSampleTime=-1  VariantActivationTime=update diagram  Latency=0  AutoFrameSizeCalculation=off
      link override Signal_Limit/_maxval: Value=KOUTP_FCM2RCErrDTC_raw32_maxval
      link override Signal_Limit/_minval: Value=KOUTP_FCM2RCErrDTC_raw32_minval
      link override Signal_Override/_ovrdflg: Value=KOUTP_FCM2RCErrDTC_raw32_ovrdflg
      link override Signal_Override/_ovrdval: Value=KOUTP_FCM2RCErrDTC_raw32_ovrdval
  VDDM_FCM3CSErrDTC_raw32_Inproc : FVT_lib/outp/OverrideAndLimit  SystemSampleTime=-1  VariantActivationTime=update diagram  Latency=0  AutoFrameSizeCalculation=off
      link override Signal_Limit/_maxval: Value=KOUTP_FCM3CSErrDTC_raw32_maxval
      link override Signal_Limit/_minval: Value=KOUTP_FCM3CSErrDTC_raw32_minval
      link override Signal_Override/_ovrdflg: Value=KOUTP_FCM3CSErrDTC_raw32_ovrdflg
      link override Signal_Override/_ovrdval: Value=KOUTP_FCM3CSErrDTC_raw32_ovrdval
  VDDM_FCM3NoComDTC_raw32_Inproc : FVT_lib/outp/OverrideAndLimit  SystemSampleTime=-1  VariantActivationTime=update diagram  Latency=0  AutoFrameSizeCalculation=off
      link override Signal_Limit/_maxval: Value=KOUTP_FCM3NoComDTC_raw32_maxval
      link override Signal_Limit/_minval: Value=KOUTP_FCM3NoComDTC_raw32_minval
      link override Signal_Override/_ovrdflg: Value=KOUTP_FCM3NoComDTC_raw32_ovrdflg
      link override Signal_Override/_ovrdval: Value=KOUTP_FCM3NoComDTC_raw32_ovrdval
  VDDM_FCM3RCErrDTC_raw32_Inproc : FVT_lib/outp/OverrideAndLimit  SystemSampleTime=-1  VariantActivationTime=update diagram  Latency=0  AutoFrameSizeCalculation=off
      link override Signal_Limit/_maxval: Value=KOUTP_FCM3RCErrDTC_raw32_maxval
      link override Signal_Limit/_minval: Value=KOUTP_FCM3RCErrDTC_raw32_minval
      link override Signal_Override/_ovrdflg: Value=KOUTP_FCM3RCErrDTC_raw32_ovrdflg
      link override Signal_Override/_ovrdval: Value=KOUTP_FCM3RCErrDTC_raw32_ovrdval
  VDDM_FCM4CSErrDTC_raw32_Inproc : FVT_lib/outp/OverrideAndLimit  SystemSampleTime=-1  VariantActivationTime=update diagram  Latency=0  AutoFrameSizeCalculation=off
      link override Signal_Limit/_maxval: Value=KOUTP_FCM4CSErrDTC_raw32_maxval
      link override Signal_Limit/_minval: Value=KOUTP_FCM4CSErrDTC_raw32_minval
      link override Signal_Override/_ovrdflg: Value=KOUTP_FCM4CSErrDTC_raw32_ovrdflg
      link override Signal_Override/_ovrdval: Value=KOUTP_FCM4CSErrDTC_raw32_ovrdval
  VDDM_FCM4NoComDTC_raw32_Inproc : FVT_lib/outp/OverrideAndLimit  SystemSampleTime=-1  VariantActivationTime=update diagram  Latency=0  AutoFrameSizeCalculation=off
      link override Signal_Limit/_maxval: Value=KOUTP_FCM4NoComDTC_raw32_maxval
      link override Signal_Limit/_minval: Value=KOUTP_FCM4NoComDTC_raw32_minval
      link override Signal_Override/_ovrdflg: Value=KOUTP_FCM4NoComDTC_raw32_ovrdflg
      link override Signal_Override/_ovrdval: Value=KOUTP_FCM4NoComDTC_raw32_ovrdval
  VDDM_FCM5CSErrDTC_raw32_Inproc : FVT_lib/outp/OverrideAndLimit  SystemSampleTime=-1  VariantActivationTime=update diagram  Latency=0  AutoFrameSizeCalculation=off
      link override Signal_Limit/_maxval: Value=KOUTP_FCM5CSErrDTC_raw32_maxval
      link override Signal_Limit/_minval: Value=KOUTP_FCM5CSErrDTC_raw32_minval
      link override Signal_Override/_ovrdflg: Value=KOUTP_FCM5CSErrDTC_raw32_ovrdflg
      link override Signal_Override/_ovrdval: Value=KOUTP_FCM5CSErrDTC_raw32_ovrdval
  VDDM_FCM5NoComDTC_raw32_Inproc : FVT_lib/outp/OverrideAndLimit  SystemSampleTime=-1  VariantActivationTime=update diagram  Latency=0  AutoFrameSizeCalculation=off
      link override Signal_Limit/_maxval: Value=KOUTP_FCM5NoComDTC_raw32_maxval
      link override Signal_Limit/_minval: Value=KOUTP_FCM5NoComDTC_raw32_minval
      link override Signal_Override/_ovrdflg: Value=KOUTP_FCM5NoComDTC_raw32_ovrdflg
      link override Signal_Override/_ovrdval: Value=KOUTP_FCM5NoComDTC_raw32_ovrdval
  VDDM_FCMACCSigErrDetDTC_raw32_Inproc : FVT_lib/outp/OverrideAndLimit  SystemSampleTime=-1  VariantActivationTime=update diagram  Latency=0  AutoFrameSizeCalculation=off
      link override Signal_Limit/_maxval: Value=KOUTP_FCMACCSigErrDetDTC_raw32_maxval
      link override Signal_Limit/_minval: Value=KOUTP_FCMACCSigErrDetDTC_raw32_minval
      link override Signal_Override/_ovrdflg: Value=KOUTP_FCMACCSigErrDetDTC_raw32_ovrdflg
      link override Signal_Override/_ovrdval: Value=KOUTP_FCMACCSigErrDetDTC_raw32_ovrdval
  VDDM_FCRUSSDTC_raw32_Inproc : FVT_lib/outp/OverrideAndLimit  SystemSampleTime=-1  VariantActivationTime=update diagram  Latency=0  AutoFrameSizeCalculation=off
      link override Signal_Limit/_maxval: Value=KOUTP_FCRUSSDTC_raw32_maxval
      link override Signal_Limit/_minval: Value=KOUTP_FCRUSSDTC_raw32_minval
      link override Signal_Override/_ovrdflg: Value=KOUTP_FCRUSSDTC_raw32_ovrdflg
      link override Signal_Override/_ovrdval: Value=KOUTP_FCRUSSDTC_raw32_ovrdval
  VDDM_FLDoorSWDTC_raw32_Inproc : FVT_lib/outp/OverrideAndLimit  SystemSampleTime=-1  VariantActivationTime=update diagram  Latency=0  AutoFrameSizeCalculation=off
      link override Signal_Limit/_maxval: Value=KOUTP_FLDoorSWDTC_raw32_maxval
      link override Signal_Limit/_minval: Value=KOUTP_FLDoorSWDTC_raw32_minval
      link override Signal_Override/_ovrdflg: Value=KOUTP_FLDoorSWDTC_raw32_ovrdflg
      link override Signal_Override/_ovrdval: Value=KOUTP_FLDoorSWDTC_raw32_ovrdval
  VDDM_FLLUSSDTC_raw32_Inproc : FVT_lib/outp/OverrideAndLimit  SystemSampleTime=-1  VariantActivationTime=update diagram  Latency=0  AutoFrameSizeCalculation=off
      link override Signal_Limit/_maxval: Value=KOUTP_FLLUSSDTC_raw32_maxval
      link override Signal_Limit/_minval: Value=KOUTP_FLLUSSDTC_raw32_minval
      link override Signal_Override/_ovrdflg: Value=KOUTP_FLLUSSDTC_raw32_ovrdflg
      link override Signal_Override/_ovrdval: Value=KOUTP_FLLUSSDTC_raw32_ovrdval
  VDDM_FLRUSSDTC_raw32_Inproc : FVT_lib/outp/OverrideAndLimit  SystemSampleTime=-1  VariantActivationTime=update diagram  Latency=0  AutoFrameSizeCalculation=off
      link override Signal_Limit/_maxval: Value=KOUTP_FLRUSSDTC_raw32_maxval
      link override Signal_Limit/_minval: Value=KOUTP_FLRUSSDTC_raw32_minval
      link override Signal_Override/_ovrdflg: Value=KOUTP_FLRUSSDTC_raw32_ovrdflg
      link override Signal_Override/_ovrdval: Value=KOUTP_FLRUSSDTC_raw32_ovrdval
  VDDM_FMLUSSDTC_raw32_Inproc : FVT_lib/outp/OverrideAndLimit  SystemSampleTime=-1  VariantActivationTime=update diagram  Latency=0  AutoFrameSizeCalculation=off
      link override Signal_Limit/_maxval: Value=KOUTP_FMLUSSDTC_raw32_maxval
      link override Signal_Limit/_minval: Value=KOUTP_FMLUSSDTC_raw32_minval
      link override Signal_Override/_ovrdflg: Value=KOUTP_FMLUSSDTC_raw32_ovrdflg
      link override Signal_Override/_ovrdval: Value=KOUTP_FMLUSSDTC_raw32_ovrdval
  VDDM_FMRUSSDTC_raw32_Inproc : FVT_lib/outp/OverrideAndLimit  SystemSampleTime=-1  VariantActivationTime=update diagram  Latency=0  AutoFrameSizeCalculation=off
      link override Signal_Limit/_maxval: Value=KOUTP_FMRUSSDTC_raw32_maxval
      link override Signal_Limit/_minval: Value=KOUTP_FMRUSSDTC_raw32_minval
      link override Signal_Override/_ovrdflg: Value=KOUTP_FMRUSSDTC_raw32_ovrdflg
      link override Signal_Override/_ovrdval: Value=KOUTP_FMRUSSDTC_raw32_ovrdval
  VDDM_FRDoorSWDTC_raw32_Inproc : FVT_lib/outp/OverrideAndLimit  SystemSampleTime=-1  VariantActivationTime=update diagram  Latency=0  AutoFrameSizeCalculation=off
      link override Signal_Limit/_maxval: Value=KOUTP_FRDoorSWDTC_raw32_maxval
      link override Signal_Limit/_minval: Value=KOUTP_FRDoorSWDTC_raw32_minval
      link override Signal_Override/_ovrdflg: Value=KOUTP_FRDoorSWDTC_raw32_ovrdflg
      link override Signal_Override/_ovrdval: Value=KOUTP_FRDoorSWDTC_raw32_ovrdval
  VDDM_FrMCUSigErrDetDTC_raw32_Inproc : FVT_lib/outp/OverrideAndLimit  SystemSampleTime=-1  VariantActivationTime=update diagram  Latency=0  AutoFrameSizeCalculation=off
      link override Signal_Limit/_maxval: Value=KOUTP_FrMCUSigErrDetDTC_raw32_maxval
      link override Signal_Limit/_minval: Value=KOUTP_FrMCUSigErrDetDTC_raw32_minval
      link override Signal_Override/_ovrdflg: Value=KOUTP_FrMCUSigErrDetDTC_raw32_ovrdflg
      link override Signal_Override/_ovrdval: Value=KOUTP_FrMCUSigErrDetDTC_raw32_ovrdval
  VDDM_FrMCUTqErrDTC_raw32_Inproc : FVT_lib/outp/OverrideAndLimit  SystemSampleTime=-1  VariantActivationTime=update diagram  Latency=0  AutoFrameSizeCalculation=off
      link override Signal_Limit/_maxval: Value=KOUTP_FrMCUTqErrDTC_raw32_maxval
      link override Signal_Limit/_minval: Value=KOUTP_FrMCUTqErrDTC_raw32_minval
      link override Signal_Override/_ovrdflg: Value=KOUTP_FrMCUTqErrDTC_raw32_ovrdflg
      link override Signal_Override/_ovrdval: Value=KOUTP_FrMCUTqErrDTC_raw32_ovrdval
  VDDM_HVB4PreDTC_raw32_Inproc : FVT_lib/outp/OverrideAndLimit  SystemSampleTime=-1  VariantActivationTime=update diagram  Latency=0  AutoFrameSizeCalculation=off
      link override Signal_Limit/_maxval: Value=KOUTP_HVB4PreDTC_raw32_maxval
      link override Signal_Limit/_minval: Value=KOUTP_HVB4PreDTC_raw32_minval
      link override Signal_Override/_ovrdflg: Value=KOUTP_HVB4PreDTC_raw32_ovrdflg
      link override Signal_Override/_ovrdval: Value=KOUTP_HVB4PreDTC_raw32_ovrdval
  VDDM_HVRlyCloDTC_raw32_Inproc : FVT_lib/outp/OverrideAndLimit  SystemSampleTime=-1  VariantActivationTime=update diagram  Latency=0  AutoFrameSizeCalculation=off
      link override Signal_Limit/_maxval: Value=KOUTP_HVRlyCloDTC_raw32_maxval
      link override Signal_Limit/_minval: Value=KOUTP_HVRlyCloDTC_raw32_minval
      link override Signal_Override/_ovrdflg: Value=KOUTP_HVRlyCloDTC_raw32_ovrdflg
      link override Signal_Override/_ovrdval: Value=KOUTP_HVRlyCloDTC_raw32_ovrdval
  VDDM_HVRlyOpDTC_raw32_Inproc : FVT_lib/outp/OverrideAndLimit  SystemSampleTime=-1  VariantActivationTime=update diagram  Latency=0  AutoFrameSizeCalculation=off
      link override Signal_Limit/_maxval: Value=KOUTP_HVRlyOpDTC_raw32_maxval
      link override Signal_Limit/_minval: Value=KOUTP_HVRlyOpDTC_raw32_minval
      link override Signal_Override/_ovrdflg: Value=KOUTP_HVRlyOpDTC_raw32_ovrdflg
      link override Signal_Override/_ovrdval: Value=KOUTP_HVRlyOpDTC_raw32_ovrdval
  VDDM_HVRlyOpFail_flg_Inproc : FVT_lib/outp/OverrideAndLimit  SystemSampleTime=-1  VariantActivationTime=update diagram  Latency=0  AutoFrameSizeCalculation=off
      link override Signal_Limit/_maxval: Value=KOUTP_HVRlyOpFail_flg_maxval
      link override Signal_Limit/_minval: Value=KOUTP_HVRlyOpFail_flg_minval
      link override Signal_Override/_ovrdflg: Value=KOUTP_HVRlyOpFail_flg_ovrdflg
      link override Signal_Override/_ovrdval: Value=KOUTP_HVRlyOpFail_flg_ovrdval
  VDDM_HiLvSaChkDTC_raw32_Inproc : FVT_lib/outp/OverrideAndLimit  SystemSampleTime=-1  VariantActivationTime=update diagram  Latency=0  AutoFrameSizeCalculation=off
      link override Signal_Limit/_maxval: Value=KOUTP_HiLvSaChkDTC_raw32_maxval
      link override Signal_Limit/_minval: Value=KOUTP_HiLvSaChkDTC_raw32_minval
      link override Signal_Override/_ovrdflg: Value=KOUTP_HiLvSaChkDTC_raw32_ovrdflg
      link override Signal_Override/_ovrdval: Value=KOUTP_HiLvSaChkDTC_raw32_ovrdval
  VDDM_HoodSWDTC_raw32_Inproc : FVT_lib/outp/OverrideAndLimit  SystemSampleTime=-1  VariantActivationTime=update diagram  Latency=0  AutoFrameSizeCalculation=off
      link override Signal_Limit/_maxval: Value=KOUTP_HoodSWDTC_raw32_maxval
      link override Signal_Limit/_minval: Value=KOUTP_HoodSWDTC_raw32_minval
      link override Signal_Override/_ovrdflg: Value=KOUTP_HoodSWDTC_raw32_ovrdflg
      link override Signal_Override/_ovrdval: Value=KOUTP_HoodSWDTC_raw32_ovrdval
  VDDM_ISAMalfuncDetDTC_raw32_Inproc : FVT_lib/outp/OverrideAndLimit  SystemSampleTime=-1  VariantActivationTime=update diagram  Latency=0  AutoFrameSizeCalculation=off
      link override Signal_Limit/_maxval: Value=KOUTP_ISAMalfuncDetDTC_raw32_maxval
      link override Signal_Limit/_minval: Value=KOUTP_ISAMalfuncDetDTC_raw32_minval
      link override Signal_Override/_ovrdflg: Value=KOUTP_ISAMalfuncDetDTC_raw32_ovrdflg
      link override Signal_Override/_ovrdval: Value=KOUTP_ISAMalfuncDetDTC_raw32_ovrdval
  VDDM_IniLVLoDTC_raw32_Inproc : FVT_lib/outp/OverrideAndLimit  SystemSampleTime=-1  VariantActivationTime=update diagram  Latency=0  AutoFrameSizeCalculation=off
      link override Signal_Limit/_maxval: Value=KOUTP_IniLVLoDTC_raw32_maxval
      link override Signal_Limit/_minval: Value=KOUTP_IniLVLoDTC_raw32_minval
      link override Signal_Override/_ovrdflg: Value=KOUTP_IniLVLoDTC_raw32_ovrdflg
      link override Signal_Override/_ovrdval: Value=KOUTP_IniLVLoDTC_raw32_ovrdval
  VDDM_KeyAuthDTC_raw32_Inproc : FVT_lib/outp/OverrideAndLimit  SystemSampleTime=-1  VariantActivationTime=update diagram  Latency=0  AutoFrameSizeCalculation=off
      link override Signal_Limit/_maxval: Value=KOUTP_KeyAuthDTC_raw32_maxval
      link override Signal_Limit/_minval: Value=KOUTP_KeyAuthDTC_raw32_minval
      link override Signal_Override/_ovrdflg: Value=KOUTP_KeyAuthDTC_raw32_ovrdflg
      link override Signal_Override/_ovrdval: Value=KOUTP_KeyAuthDTC_raw32_ovrdval
  VDDM_LFBatwarnDTC_raw32_Inproc : FVT_lib/outp/OverrideAndLimit  SystemSampleTime=-1  VariantActivationTime=update diagram  Latency=0  AutoFrameSizeCalculation=off
      link override Signal_Limit/_maxval: Value=KOUTP_LFBatwarnDTC_raw32_maxval
      link override Signal_Limit/_minval: Value=KOUTP_LFBatwarnDTC_raw32_minval
      link override Signal_Override/_ovrdflg: Value=KOUTP_LFBatwarnDTC_raw32_ovrdflg
      link override Signal_Override/_ovrdval: Value=KOUTP_LFBatwarnDTC_raw32_ovrdval
  VDDM_LFPressIndiDTC_raw32_Inproc : FVT_lib/outp/OverrideAndLimit  SystemSampleTime=-1  VariantActivationTime=update diagram  Latency=0  AutoFrameSizeCalculation=off
      link override Signal_Limit/_maxval: Value=KOUTP_LFPressIndiDTC_raw32_maxval
      link override Signal_Limit/_minval: Value=KOUTP_LFPressIndiDTC_raw32_minval
      link override Signal_Override/_ovrdflg: Value=KOUTP_LFPressIndiDTC_raw32_ovrdflg
      link override Signal_Override/_ovrdval: Value=KOUTP_LFPressIndiDTC_raw32_ovrdval
  VDDM_LFSensorFailDTC_raw32_Inproc : FVT_lib/outp/OverrideAndLimit  SystemSampleTime=-1  VariantActivationTime=update diagram  Latency=0  AutoFrameSizeCalculation=off
      link override Signal_Limit/_maxval: Value=KOUTP_LFSensorFailDTC_raw32_maxval
      link override Signal_Limit/_minval: Value=KOUTP_LFSensorFailDTC_raw32_minval
      link override Signal_Override/_ovrdflg: Value=KOUTP_LFSensorFailDTC_raw32_ovrdflg
      link override Signal_Override/_ovrdval: Value=KOUTP_LFSensorFailDTC_raw32_ovrdval
  VDDM_LFWheelTmpHighDTC_raw32_Inproc : FVT_lib/outp/OverrideAndLimit  SystemSampleTime=-1  VariantActivationTime=update diagram  Latency=0  AutoFrameSizeCalculation=off
      link override Signal_Limit/_maxval: Value=KOUTP_LFWheelTmpHighDTC_raw32_maxval
      link override Signal_Limit/_minval: Value=KOUTP_LFWheelTmpHighDTC_raw32_minval
      link override Signal_Override/_ovrdflg: Value=KOUTP_LFWheelTmpHighDTC_raw32_ovrdflg
      link override Signal_Override/_ovrdval: Value=KOUTP_LFWheelTmpHighDTC_raw32_ovrdval
  VDDM_LRBatwarnDTC_raw32_Inproc : FVT_lib/outp/OverrideAndLimit  SystemSampleTime=-1  VariantActivationTime=update diagram  Latency=0  AutoFrameSizeCalculation=off
      link override Signal_Limit/_maxval: Value=KOUTP_LRBatwarnDTC_raw32_maxval
      link override Signal_Limit/_minval: Value=KOUTP_LRBatwarnDTC_raw32_minval
      link override Signal_Override/_ovrdflg: Value=KOUTP_LRBatwarnDTC_raw32_ovrdflg
      link override Signal_Override/_ovrdval: Value=KOUTP_LRBatwarnDTC_raw32_ovrdval
  VDDM_LRPressIndiDTC_raw32_Inproc : FVT_lib/outp/OverrideAndLimit  SystemSampleTime=-1  VariantActivationTime=update diagram  Latency=0  AutoFrameSizeCalculation=off
      link override Signal_Limit/_maxval: Value=KOUTP_LRPressIndiDTC_raw32_maxval
      link override Signal_Limit/_minval: Value=KOUTP_LRPressIndiDTC_raw32_minval
      link override Signal_Override/_ovrdflg: Value=KOUTP_LRPressIndiDTC_raw32_ovrdflg
      link override Signal_Override/_ovrdval: Value=KOUTP_LRPressIndiDTC_raw32_ovrdval
  VDDM_LRSensorFailDTC_raw32_Inproc : FVT_lib/outp/OverrideAndLimit  SystemSampleTime=-1  VariantActivationTime=update diagram  Latency=0  AutoFrameSizeCalculation=off
      link override Signal_Limit/_maxval: Value=KOUTP_LRSensorFailDTC_raw32_maxval
      link override Signal_Limit/_minval: Value=KOUTP_LRSensorFailDTC_raw32_minval
      link override Signal_Override/_ovrdflg: Value=KOUTP_LRSensorFailDTC_raw32_ovrdflg
      link override Signal_Override/_ovrdval: Value=KOUTP_LRSensorFailDTC_raw32_ovrdval
  VDDM_LRWheelTmpHighDTC_raw32_Inproc : FVT_lib/outp/OverrideAndLimit  SystemSampleTime=-1  VariantActivationTime=update diagram  Latency=0  AutoFrameSizeCalculation=off
      link override Signal_Limit/_maxval: Value=KOUTP_LRWheelTmpHighDTC_raw32_maxval
      link override Signal_Limit/_minval: Value=KOUTP_LRWheelTmpHighDTC_raw32_minval
      link override Signal_Override/_ovrdflg: Value=KOUTP_LRWheelTmpHighDTC_raw32_ovrdflg
      link override Signal_Override/_ovrdval: Value=KOUTP_LRWheelTmpHighDTC_raw32_ovrdval
  VDDM_LVSupHiDTC_raw32_Inproc : FVT_lib/outp/OverrideAndLimit  SystemSampleTime=-1  VariantActivationTime=update diagram  Latency=0  AutoFrameSizeCalculation=off
      link override Signal_Limit/_maxval: Value=KOUTP_LVSupHiDTC_raw32_maxval
      link override Signal_Limit/_minval: Value=KOUTP_LVSupHiDTC_raw32_minval
      link override Signal_Override/_ovrdflg: Value=KOUTP_LVSupHiDTC_raw32_ovrdflg
      link override Signal_Override/_ovrdval: Value=KOUTP_LVSupHiDTC_raw32_ovrdval
  VDDM_LVSupLoDTC_raw32_Inproc : FVT_lib/outp/OverrideAndLimit  SystemSampleTime=-1  VariantActivationTime=update diagram  Latency=0  AutoFrameSizeCalculation=off
      link override Signal_Limit/_maxval: Value=KOUTP_LVSupLoDTC_raw32_maxval
      link override Signal_Limit/_minval: Value=KOUTP_LVSupLoDTC_raw32_minval
      link override Signal_Override/_ovrdflg: Value=KOUTP_LVSupLoDTC_raw32_ovrdflg
      link override Signal_Override/_ovrdval: Value=KOUTP_LVSupLoDTC_raw32_ovrdval
  VDDM_LVSysErrPwrOutErr_flg_Inproc : FVT_lib/outp/OverrideAndLimit  SystemSampleTime=-1  VariantActivationTime=update diagram  Latency=0  AutoFrameSizeCalculation=off
      link override Signal_Limit/_maxval: Value=KOUTP_LVSysErrPwrOutErr_flg_maxval
      link override Signal_Limit/_minval: Value=KOUTP_LVSysErrPwrOutErr_flg_minval
      link override Signal_Override/_ovrdflg: Value=KOUTP_LVSysErrPwrOutErr_flg_ovrdflg
      link override Signal_Override/_ovrdval: Value=KOUTP_LVSysErrPwrOutErr_flg_ovrdval
  VDDM_LimpHomeActTmp_flg_Inproc : FVT_lib/outp/OverrideAndLimit  SystemSampleTime=-1  VariantActivationTime=update diagram  Latency=0  AutoFrameSizeCalculation=off
      link override Signal_Limit/_maxval: Value=KOUTP_LimpHomeActTmp_flg_maxval
